simulink model "Production_ToBe_batched_upgrade1_run2026"  (R2025b)
settings: Solver=VariableStepAuto  StartTime=0.0  StopTime=105600  RelTol=1e-3
undefined symbols (not defined in the file or in its folder): m, n
(part 1 of 2)
settings Model: Creator=MSI  LastModifiedBy=MSI

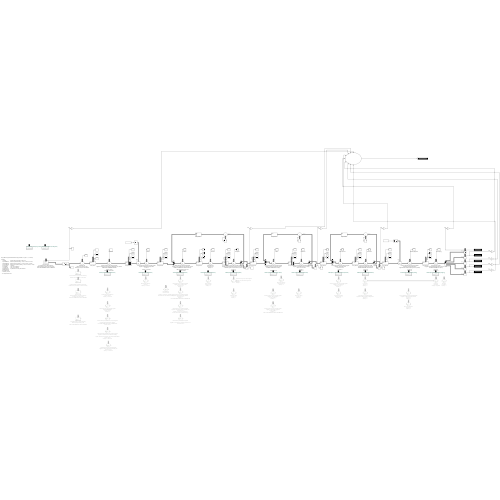
[thumbnail: Simulink's stored preview of the top-level diagram]
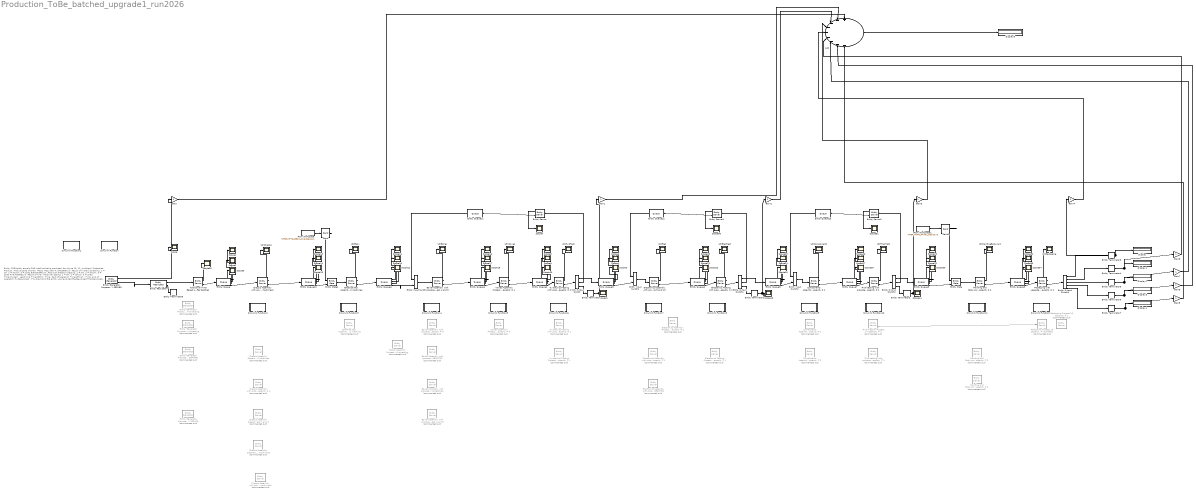
== system Production_ToBe_batched_upgrade1_run2026 ==
  note: Entity (ONE entity equals ONE machine being produced, be it type 10, 11, or others.)
      |
      | Properties:
      | Product : Product code of entity (PC10, PC11 etc)
      | HydTestResult : Result of hydraulics testing. 1 = OK, 2 = rework, 3 = scrap
      | ElecTestResult : Result of electronic testing. 1 = OK, 2 = rework, 3 = scrap
      | FinalTestResult : Result of final (machine) testing. 1 = OK, 2 = rework, 3 = scrap
      | TimeinSytem : Lead time
      | TimeAtStart : Time, start of operation
      | TimeAtFinish : Time, end of operation
      | HydReworked : If hydraulics of the entity was reworked
      | ElecReworked
      | FinalReworked
      | Endtime, process
      | TTP, process for each
  Add : Sum  Inputs=+--------
  Additional Time Based on the last entity type Models the setup time after batches : EntityServer  InputPortMessageModes=m  OutputPortMessageModes=n,m  Capacity=1  ServiceTimeSource=MATLAB action  ServiceTimeAction=|  Utilization=on
      | % Since this server is a proxy, dt = 0
      | dt = 0;
      | 
      | % Setup times
      | persistent last_product;
      | 
      | if isempty(last_product)
      |     last_product = 0;
      | end
      | 
      | setuptime = 0;
      | 
      | if last_product == 0
      |     % First entity - no setup time needed
      |     setuptime = 0;
      | elseif last_product ~= entity.Product
      |     % Product change detected - apply setup time based on previous product
      |     if last_product == 1
      |         setuptime = 0;
      |     elseif last_product == 2
      |         setuptime = 0;
      |     elseif last_product == 3
      |         setuptime = 15;
      |     elseif last_product == 4
      |         setuptime = 30;
      |     else
      |         setuptime = 35;
      |     end
      | end
      | 
      | dt = dt + setuptime;
      | last_product = entity.Product;
      settings: OutputPortMap=o5,o9
  "Boiler Assembly Process 4 and 5 Capacity = 3 machines, operated by 3 Rework decision after hydraulics testing" : EntityServer  Commented=on  InputPortMessageModes=m  OutputPortMessageModes=n,m  Capacity=3  ServiceTimeSource=MATLAB action  ServiceTimeAction=|  ServiceCompleteAction=|  Utilization=on
      ServiceTimeAction=|
      | % Main action of the server. Which means, this code explains what the entity department should be doing
      | % Assign entity processing times based on the time listed on the spreadsheet
      | % For process 4 and 5
      | 
      | generateTime = @(mu, cv) lognrnd(log(mu) - 0.5*log(1+cv^2), sqrt(log(1+cv^2)));
      | 
      | if entity.HydReworked == 1;
      |     dt = 1;
      | else
      |     if entity.Product == 1 | entity.Product == 3
      |     dt = generateTime(20.4, 1) + generateTime(19.9, 1);
      |     elseif entity.Product == 2 | entity.Product == 4 | entity.Product == 5
      |     dt = generateTime(28.2, 1) + generateTime (19.9, 1);
      |     else
      |     dt = 0; 
      |     end
      | end
      | 
      | % Setup times
      | persistent last_product;
      | 
      | if isempty(last_product)
      |     last_product = 0;
      | end
      | 
      | setuptime = 0;
      | 
      | if last_product == 0
      |     % First entity - no setup time needed
      |     setuptime = 0;
      | elseif last_product ~= entity.Product
      |     % Product change detected - apply setup time based on previous product
      |     if last_product == 1
      |         setuptime = 3;
      |     elseif last_product == 2
      |         setuptime = 4;
      |     elseif last_product == 3
      |         setuptime = 3;
      |     elseif last_product == 4
      |         setuptime = 4;
      |     else
      |         setuptime = 4;
      |     end
      | end
      | 
      | dt = dt + setuptime;
      | last_product = entity.Product;
      ServiceCompleteAction=|
      | % Define persistent variables to track the total throughput time and entity count
      | persistent TTPtotal entityCount;
      | % TTPtotal = tracks the total TTP of the system. In which, when every new station is visited, the time is added
      | % entityCount =
      | 
      | % Initialize the persistent variables if they are empty
      | if isempty(TTPtotal)
      |     TTPtotal = 0;
      | end
      | if isempty(entityCount)
      |     entityCount = 0;
      | end
      | 
      | % Read the current entity's final time
      | entity.EndTimeBoiler = ReadTime();
      | 
      | % Calculate the TTP for the chassis department for the specific entity
      | % INCLUDES wait time
      | entity.TTPboiler = abs(entity.EndTimeBoiler - entity.EndTimeEbox);
      | 
      | % Update the total throughput time and entity count
      | % This is done AFTER the process, 
      |     % to mark that the entity has gone through the chassis department 
      |         % (thus TTPchassis being added)
      |             % and add that the entity, for each entity after being processed
      |             
      | TTPtotal = TTPtotal + entity.TTPboiler;
      | entityCount = entityCount + 1;
      | 
      | % Calculate the average throughput time for the chassis department
      | avgTTPboiler = TTPtotal / entityCount;
      | 
      | % Send the average throughput time to the workspace
      | ToWorkspace_Boiler(avgTTPboiler);
      settings: OutputPortMap=o5,o9
  Boiler Assembly with proposed upgrade Upgrade = AR based assembly assistant Process 4 and 5 Capacity = 1 HAS TO BE PAIRED WITH ENTITY GENERATOR : EntityServer  Commented=on  InputPortMessageModes=m  OutputPortMessageModes=n,m  Capacity=3  ServiceTimeSource=MATLAB action  ServiceTimeAction=|  ServiceCompleteAction=|  Utilization=on
      ServiceTimeAction=|
      | % Main action of the server. Which means, this code explains what the entity department should be doing
      | % Assign entity processing times based on the time listed on the spreadsheet
      | % For process 4 and 5
      | 
      | generateTime = @(mu, cv) lognrnd(log(mu) - 0.5*log(1+cv^2), sqrt(log(1+cv^2)));
      | 
      | if entity.HydReworked == 1;
      |     dt = 1;
      | else
      |     if entity.Product == 10 | entity.Product == 11
      |     dt = generateTime(20.4, 1) + generateTime(19.9, 1);
      |     dt = dt * 0.9;
      |     elseif entity.Product == 20 | entity.Product == 21 | entity.Product == 35
      |     dt = generateTime(28.2, 1) + generateTime (19.9, 1);
      |     dt = dt * 0.9;
      |     else
      |     dt = 0; 
      |     end
      | end
      ServiceCompleteAction=|
      | % Define persistent variables to track the total throughput time and entity count
      | persistent TTPtotal entityCount;
      | % TTPtotal = tracks the total TTP of the system. In which, when every new station is visited, the time is added
      | % entityCount =
      | 
      | % Initialize the persistent variables if they are empty
      | if isempty(TTPtotal)
      |     TTPtotal = 0;
      | end
      | if isempty(entityCount)
      |     entityCount = 0;
      | end
      | 
      | % Read the current entity's final time
      | entity.EndTimeBoiler = ReadTime();
      | 
      | % Calculate the TTP for the chassis department for the specific entity
      | % INCLUDES wait time
      | entity.TTPboiler = abs(entity.EndTimeBoiler - entity.EndTimeEbox);
      | 
      | % Update the total throughput time and entity count
      | % This is done AFTER the process, 
      |     % to mark that the entity has gone through the chassis department 
      |         % (thus TTPchassis being added)
      |             % and add that the entity, for each entity after being processed
      |             
      | TTPtotal = TTPtotal + entity.TTPboiler;
      | entityCount = entityCount + 1;
      | 
      | % Calculate the average throughput time for the chassis department
      | avgTTPboiler = TTPtotal / entityCount;
      | 
      | % Send the average throughput time to the workspace
      | ToWorkspace_Boiler(avgTTPboiler);
      settings: OutputPortMap=o5,o9
  "Boiler Assembly with proposed upgrade Upgrade = Automated pressure regulation tool Process 4 and 5 Capacity = 3 machines, operated by 3 Rework decision after hydraulics testing1" : EntityServer  Commented=on  InputPortMessageModes=m  OutputPortMessageModes=n,m  Capacity=3  ServiceTimeSource=MATLAB action  ServiceTimeAction=|  ServiceCompleteAction=|  Utilization=on
      ServiceTimeAction=|
      | % Main action of the server. Which means, this code explains what the entity department should be doing
      | % Assign entity processing times based on the time listed on the spreadsheet
      | % For process 4 and 5
      | 
      | generateTime = @(mu, cv) lognrnd(log(mu) - 0.5*log(1+cv^2), sqrt(log(1+cv^2)));
      | 
      | if entity.HydReworked == 1;
      |     dt = 1;
      | else
      |     if entity.Product == 10 | entity.Product == 11
      |     dt = generateTime(20.4, 1) + generateTime(19.9, 1);
      |     dt = dt * 0.95;
      |     elseif entity.Product == 20 | entity.Product == 21 | entity.Product == 35
      |     dt = generateTime(28.2, 1) + generateTime (19.9, 1);
      |     dt = dt * 0.95;
      |     else
      |     dt = 0; 
      |     end
      | end
      ServiceCompleteAction=|
      | % Define persistent variables to track the total throughput time and entity count
      | persistent TTPtotal entityCount;
      | % TTPtotal = tracks the total TTP of the system. In which, when every new station is visited, the time is added
      | % entityCount =
      | 
      | % Initialize the persistent variables if they are empty
      | if isempty(TTPtotal)
      |     TTPtotal = 0;
      | end
      | if isempty(entityCount)
      |     entityCount = 0;
      | end
      | 
      | % Read the current entity's final time
      | entity.EndTimeBoiler = ReadTime();
      | 
      | % Calculate the TTP for the chassis department for the specific entity
      | % INCLUDES wait time
      | entity.TTPboiler = abs(entity.EndTimeBoiler - entity.EndTimeEbox);
      | 
      | % Update the total throughput time and entity count
      | % This is done AFTER the process, 
      |     % to mark that the entity has gone through the chassis department 
      |         % (thus TTPchassis being added)
      |             % and add that the entity, for each entity after being processed
      |             
      | TTPtotal = TTPtotal + entity.TTPboiler;
      | entityCount = entityCount + 1;
      | 
      | % Calculate the average throughput time for the chassis department
      | avgTTPboiler = TTPtotal / entityCount;
      | 
      | % Send the average throughput time to the workspace
      | ToWorkspace_Boiler(avgTTPboiler);
      settings: OutputPortMap=o5,o9
  Boiler Assembly with proposed upgrade Upgrade = Boiler insertion robot Process 4 and 5 Capacity = 3 : EntityServer  Commented=on  InputPortMessageModes=m  OutputPortMessageModes=n,m  Capacity=3  ServiceTimeSource=MATLAB action  ServiceTimeAction=|  ServiceCompleteAction=|  Utilization=on
      ServiceTimeAction=|
      | % Main action of the server. Which means, this code explains what the entity department should be doing
      | % Assign entity processing times based on the time listed on the spreadsheet
      | % For process 4 and 5
      | 
      | generateTime = @(mu, cv) lognrnd(log(mu) - 0.5*log(1+cv^2), sqrt(log(1+cv^2)));
      | 
      | if entity.HydReworked == 1;
      |     dt = 1;
      | else
      |     if entity.Product == 10 | entity.Product == 11
      |     dt = (generateTime(20.4, 1)) * 0.8 + generateTime(19.9, 1);
      |     elseif entity.Product == 20 | entity.Product == 21 | entity.Product == 35
      |     dt = (generateTime(28.2, 1)) * 0.85 + generateTime (19.9, 1);
      |     else
      |     dt = 0; 
      |     end
      | end
      ServiceCompleteAction=|
      | % Define persistent variables to track the total throughput time and entity count
      | persistent TTPtotal entityCount;
      | % TTPtotal = tracks the total TTP of the system. In which, when every new station is visited, the time is added
      | % entityCount =
      | 
      | % Initialize the persistent variables if they are empty
      | if isempty(TTPtotal)
      |     TTPtotal = 0;
      | end
      | if isempty(entityCount)
      |     entityCount = 0;
      | end
      | 
      | % Read the current entity's final time
      | entity.EndTimeBoiler = ReadTime();
      | 
      | % Calculate the TTP for the chassis department for the specific entity
      | % INCLUDES wait time
      | entity.TTPboiler = abs(entity.EndTimeBoiler - entity.EndTimeEbox);
      | 
      | % Update the total throughput time and entity count
      | % This is done AFTER the process, 
      |     % to mark that the entity has gone through the chassis department 
      |         % (thus TTPchassis being added)
      |             % and add that the entity, for each entity after being processed
      |             
      | TTPtotal = TTPtotal + entity.TTPboiler;
      | entityCount = entityCount + 1;
      | 
      | % Calculate the average throughput time for the chassis department
      | avgTTPboiler = TTPtotal / entityCount;
      | 
      | % Send the average throughput time to the workspace
      | ToWorkspace_Boiler(avgTTPboiler);
      settings: OutputPortMap=o5,o9
  Boiler Assembly with proposed upgrade Upgrade = Vision-guided robot for main boiler insertion DOUBLE UPGRADE with AR based assembly TRIPLE upgrade insertion robot Process 4 and 5 : EntityServer  InputPortMessageModes=m  OutputPortMessageModes=n,m  Capacity=3  ServiceTimeSource=MATLAB action  ServiceTimeAction=|  ServiceCompleteAction=|  Utilization=on
      ServiceTimeAction=|
      | % Main action of the server. Which means, this code explains what the entity department should be doing
      | % Assign entity processing times based on the time listed on the spreadsheet
      | % For process 4 and 5
      | 
      | generateTime = @(mu, cv) lognrnd(log(mu) - 0.5*log(1+cv^2), sqrt(log(1+cv^2)));
      | 
      | if entity.HydReworked == 1;
      |     dt = 1;
      | else
      |     if entity.Product == 1 | entity.Product == 2
      |     dt = generateTime(20.4, 1) + generateTime(19.9, 1); %triple upgrade
      |     dt = dt * 0.65;
      |     elseif entity.Product == 3 | entity.Product == 4 | entity.Product == 5
      |     dt = generateTime(28.2, 1) + generateTime (19.9, 1); %triple upgrade
      |     dt = dt * 0.65;
      |     else
      |     dt = 0; 
      |     end
      | end
      | 
      | % double upgrade
      | dt = dt * 0.9;
      | 
      | 
      | % Setup times
      | persistent last_product;
      | 
      | if isempty(last_product)
      |     last_product = 0;
      | end
      | 
      | setuptime = 0;
      | 
      | if last_product == 0
      |     % First entity - no setup time needed
      |     setuptime = 0;
      | elseif last_product ~= entity.Product
      |     % Product change detected - apply setup time based on previous product
      |     if last_product == 1
      |         setuptime = 3;
      |     elseif last_product == 2
      |         setuptime = 4;
      |     elseif last_product == 3
      |         setuptime = 3;
      |     elseif last_product == 4
      |         setuptime = 4;
      |     else
      |         setuptime = 4;
      |     end
      | end
      | 
      | dt = dt + setuptime;
      | last_product = entity.Product;
      ServiceCompleteAction=|
      | % Define persistent variables to track the total throughput time and entity count
      | persistent TTPtotal entityCount;
      | % TTPtotal = tracks the total TTP of the system. In which, when every new station is visited, the time is added
      | % entityCount =
      | 
      | % Initialize the persistent variables if they are empty
      | if isempty(TTPtotal)
      |     TTPtotal = 0;
      | end
      | if isempty(entityCount)
      |     entityCount = 0;
      | end
      | 
      | % Read the current entity's final time
      | entity.EndTimeBoiler = ReadTime();
      | 
      | % Calculate the TTP for the chassis department for the specific entity
      | % INCLUDES wait time
      | entity.TTPboiler = abs(entity.EndTimeBoiler - entity.EndTimeEbox);
      | 
      | % Update the total throughput time and entity count
      | % This is done AFTER the process, 
      |     % to mark that the entity has gone through the chassis department 
      |         % (thus TTPchassis being added)
      |             % and add that the entity, for each entity after being processed
      |             
      | TTPtotal = TTPtotal + entity.TTPboiler;
      | entityCount = entityCount + 1;
      | 
      | % Calculate the average throughput time for the chassis department
      | avgTTPboiler = TTPtotal / entityCount;
      | 
      | % Send the average throughput time to the workspace
      | ToWorkspace_Boiler(avgTTPboiler);
      settings: OutputPortMap=o5,o9
  "Boiler Assembly with proposed upgrade Upgrade = extra workbench, capacity grew from 3 to 4 Process 4 and 5" : EntityServer  Commented=on  InputPortMessageModes=m  OutputPortMessageModes=n,m  Capacity=4  ServiceTimeSource=MATLAB action  ServiceTimeAction=|  ServiceCompleteAction=|  Utilization=on
      ServiceTimeAction=|
      | % Main action of the server. Which means, this code explains what the entity department should be doing
      | % Assign entity processing times based on the time listed on the spreadsheet
      | % For process 4 and 5
      | 
      | generateTime = @(mu, cv) lognrnd(log(mu) - 0.5*log(1+cv^2), sqrt(log(1+cv^2)));
      | 
      | if entity.HydReworked == 1;
      |     dt = 1;
      | else
      |     if entity.Product == 10 | entity.Product == 11
      |     dt = generateTime(20.4, 1) + generateTime(19.9, 1);
      |     elseif entity.Product == 20 | entity.Product == 21 | entity.Product == 35
      |     dt = generateTime(28.2, 1) + generateTime (19.9, 1);
      |     else
      |     dt = 0; 
      |     end
      | end
      ServiceCompleteAction=|
      | % Define persistent variables to track the total throughput time and entity count
      | persistent TTPtotal entityCount;
      | % TTPtotal = tracks the total TTP of the system. In which, when every new station is visited, the time is added
      | % entityCount =
      | 
      | % Initialize the persistent variables if they are empty
      | if isempty(TTPtotal)
      |     TTPtotal = 0;
      | end
      | if isempty(entityCount)
      |     entityCount = 0;
      | end
      | 
      | % Read the current entity's final time
      | entity.EndTimeBoiler = ReadTime();
      | 
      | % Calculate the TTP for the chassis department for the specific entity
      | % INCLUDES wait time
      | entity.TTPboiler = abs(entity.EndTimeBoiler - entity.EndTimeEbox);
      | 
      | % Update the total throughput time and entity count
      | % This is done AFTER the process, 
      |     % to mark that the entity has gone through the chassis department 
      |         % (thus TTPchassis being added)
      |             % and add that the entity, for each entity after being processed
      |             
      | TTPtotal = TTPtotal + entity.TTPboiler;
      | entityCount = entityCount + 1;
      | 
      | % Calculate the average throughput time for the chassis department
      | avgTTPboiler = TTPtotal / entityCount;
      | 
      | % Send the average throughput time to the workspace
      | ToWorkspace_Boiler(avgTTPboiler);
      settings: OutputPortMap=o5,o9
  "Chassis Assembly Departmen with proposed upgrade Upgrade = Smart fixtures wth automatic clamping Impact = Assembly time variability -50%, ONLY GROUP HEAD Process 1 and 2 Capacity = 3 machines1" : EntityServer  Commented=on  InputPortMessageModes=m  OutputPortMessageModes=n,m  Capacity=3  ServiceTimeSource=MATLAB action  ServiceTimeAction=|  ServiceCompleteAction=|  Utilization=on
      ServiceTimeAction=|
      | % Main action of the server
      | 
      | % Function to generate processing time based on mean and CV using lognormal
      | generateTime = @(mu, cv) lognrnd(log(mu) - 0.5*log(1+cv^2), sqrt(log(1+cv^2)));
      | 
      | if entity.Product == 1
      |     dt = generateTime(29.7, 0.8) + generateTime(14.7, 0.4);
      | elseif entity.Product == 2
      |     dt = generateTime(31.2, 0.8) + generateTime(14.7, 0.4);
      | elseif entity.Product == 3
      |     dt = generateTime(29.7, 0.8) + generateTime(17.6, 0.4);
      | elseif entity.Product == 4
      |     dt = generateTime(31.2, 0.8) + generateTime(17.6, 0.4);
      | elseif entity.Product == 5
      |     dt = generateTime(34.4, 0.8) + generateTime(17.6, 0.4);
      | else
      |     dt = 0; 
      | end
      | 
      | % Setup times
      | persistent last_product;
      | last_product = 0;
      | setuptime = 0;
      | if last_product == 0
      |     last_product = entity.Product;   % first entity
      |     dt = dt + setuptime;
      | else
      |     if last_product == entity.Product;
      |         dt = dt + setuptime;
      |     else
      |         if last_product ~= entity.Product
      |             if last_product == 1
      |                 setuptime = 5;
      |                 dt = dt + setuptime;
      |             elseif last_product == 2
      |                 setuptime = 6;
      |                 dt = dt + setuptime;
      |             elseif last_product == 3
      |                 setuptime = 5;
      |                 dt = dt + setuptime;
      |             elseif last_product == 4
      |                 setuptime = 6;
      |                 dt = dt + setuptime;
      |             else
      |                 setuptime = 6;
      |                 dt = dt + setuptime;
      |             end
      |         end
      |     end
      |     last_product = entity.Product;
      | end
      ServiceCompleteAction=|
      | % Define persistent variables to track the total throughput time and entity count
      | persistent TTPtotal entityCount;
      | % TTPtotal = tracks the total TTP of the system. In which, when every new station is visited, the time is added
      | % entityCount =
      | 
      | % Initialize the persistent variables if they are empty
      | if isempty(TTPtotal)
      |     TTPtotal = 0;
      | end
      | if isempty(entityCount)
      |     entityCount = 0;
      | end
      | 
      | % Read the current entity's final time
      | entity.EndTimeChassis = ReadTime();
      | 
      | % Calculate the TTP for the chassis department for the specific entity
      | % INCLUDES wait time
      | entity.TTPchassis = abs(entity.EndTimeChassis - entity.StartTime);
      | 
      | % Update the total throughput time and entity count
      | % This is done AFTER the process, 
      |     % to mark that the entity has gone through the chassis department 
      |         % (thus TTPchassis being added)
      |             % and add that the entity, for each entity after being processed
      |             
      | TTPtotal = TTPtotal + entity.TTPchassis;
      | entityCount = entityCount + 1;
      | 
      | % Calculate the average throughput time for the chassis department
      | avgTTPchassis = TTPtotal / entityCount;
      | 
      | % Send the average throughput time to the workspace
      | ToWorkspace_Chassis(avgTTPchassis);
      settings: OutputPortMap=o5,o9
  Chassis Assembly Department Process 1 and 2 Capacity = 3 machines : EntityServer  Commented=on  InputPortMessageModes=m  OutputPortMessageModes=n,m  Capacity=3  ServiceTimeSource=MATLAB action  ServiceTimeAction=|  ServiceCompleteAction=|  Utilization=on
      ServiceTimeAction=|
      | % Main action of the server
      | 
      | % Function to generate processing time based on mean and CV using lognormal
      | generateTime = @(mu, cv) lognrnd(log(mu) - 0.5*log(1+cv^2), sqrt(log(1+cv^2)));
      | 
      | if entity.Product == 1
      |     dt = generateTime(29.7, 0.8) + generateTime(14.7, 0.8);
      | elseif entity.Product == 2
      |     dt = generateTime(31.2, 0.8) + generateTime(14.7, 0.8);
      | elseif entity.Product == 3
      |     dt = generateTime(29.7, 0.8) + generateTime(17.6, 0.8);
      | elseif entity.Product == 4
      |     dt = generateTime(31.2, 0.8) + generateTime(17.6, 0.8);
      | elseif entity.Product == 5
      |     dt = generateTime(34.4, 0.8) + generateTime(17.6, 0.8);
      | else
      |     dt = 0; 
      | end
      | 
      | % Setup times
      | persistent last_product;
      | 
      | if isempty(last_product)
      |     last_product = 0;
      | end
      | 
      | setuptime = 0;
      | 
      | if last_product == 0
      |     % First entity - no setup time needed
      |     setuptime = 0;
      | elseif last_product ~= entity.Product
      |     % Product change detected - apply setup time based on previous product
      |     if last_product == 1
      |         setuptime = 5;
      |     elseif last_product == 2
      |         setuptime = 6;
      |     elseif last_product == 3
      |         setuptime = 5;
      |     elseif last_product == 4
      |         setuptime = 6;
      |     else
      |         setuptime = 6;
      |     end
      | end
      | 
      | dt = dt + setuptime;
      | last_product = entity.Product;
      ServiceCompleteAction=|
      | % Define persistent variables to track the total throughput time and entity count
      | persistent TTPtotal entityCount;
      | % TTPtotal = tracks the total TTP of the system. In which, when every new station is visited, the time is added
      | % entityCount =
      | 
      | % Initialize the persistent variables if they are empty
      | if isempty(TTPtotal)
      |     TTPtotal = 0;
      | end
      | if isempty(entityCount)
      |     entityCount = 0;
      | end
      | 
      | % Read the current entity's final time
      | entity.EndTimeChassis = ReadTime();
      | 
      | % Calculate the TTP for the chassis department for the specific entity
      | % INCLUDES wait time
      | entity.TTPchassis = abs(entity.EndTimeChassis - entity.StartTime);
      | 
      | % Update the total throughput time and entity count
      | % This is done AFTER the process, 
      |     % to mark that the entity has gone through the chassis department 
      |         % (thus TTPchassis being added)
      |             % and add that the entity, for each entity after being processed
      |             
      | TTPtotal = TTPtotal + entity.TTPchassis;
      | entityCount = entityCount + 1;
      | 
      | % Calculate the average throughput time for the chassis department
      | avgTTPchassis = TTPtotal / entityCount;
      | 
      | % Send the average throughput time to the workspace
      | ToWorkspace_Chassis(avgTTPchassis);
      settings: OutputPortMap=o5,o9
  Chassis Assembly Department with proposed upgrade Upgrade= AR based assembly assistant HAS TO BE PAIRED WITH ENTITY GENERATOR Process 1 and 2 : EntityServer  Commented=on  InputPortMessageModes=m  OutputPortMessageModes=n,m  Capacity=3  ServiceTimeSource=MATLAB action  ServiceTimeAction=|  ServiceCompleteAction=|  Utilization=on
      ServiceTimeAction=|
      | % Main action of the server
      | 
      | % Function to generate processing time based on mean and CV using lognormal
      | generateTime = @(mu, cv) lognrnd(log(mu) - 0.5*log(1+cv^2), sqrt(log(1+cv^2)));
      | 
      | if entity.Product == 10
      |     dt = generateTime(29.7, 0.8) + generateTime(14.7, 0.8);
      |     dt = dt * 0.9;
      | elseif entity.Product == 20
      |     dt = generateTime(31.2, 0.8) + generateTime(14.7, 0.8);
      |     dt = dt * 0.9;
      | elseif entity.Product == 11
      |     dt = generateTime(29.7, 0.8) + generateTime(17.6, 0.8);
      |     dt = dt * 0.9;
      | elseif entity.Product == 21
      |     dt = generateTime(31.2, 0.8) + generateTime(17.6, 0.8);
      |     dt = dt * 0.9;
      | elseif entity.Product == 35
      |     dt = generateTime(34.4, 0.8) + generateTime(17.6, 0.8);
      |     dt = dt * 0.9;
      | else
      |     dt = 0; 
      | end
      ServiceCompleteAction=|
      | % Define persistent variables to track the total throughput time and entity count
      | persistent TTPtotal entityCount;
      | % TTPtotal = tracks the total TTP of the system. In which, when every new station is visited, the time is added
      | % entityCount =
      | 
      | % Initialize the persistent variables if they are empty
      | if isempty(TTPtotal)
      |     TTPtotal = 0;
      | end
      | if isempty(entityCount)
      |     entityCount = 0;
      | end
      | 
      | % Read the current entity's final time
      | entity.EndTimeChassis = ReadTime();
      | 
      | % Calculate the TTP for the chassis department for the specific entity
      | % INCLUDES wait time
      | entity.TTPchassis = abs(entity.EndTimeChassis - entity.StartTime);
      | 
      | % Update the total throughput time and entity count
      | % This is done AFTER the process, 
      |     % to mark that the entity has gone through the chassis department 
      |         % (thus TTPchassis being added)
      |             % and add that the entity, for each entity after being processed
      |             
      | TTPtotal = TTPtotal + entity.TTPchassis;
      | entityCount = entityCount + 1;
      | 
      | % Calculate the average throughput time for the chassis department
      | avgTTPchassis = TTPtotal / entityCount;
      | 
      | % Send the average throughput time to the workspace
      | ToWorkspace_Chassis(avgTTPchassis);
      settings: OutputPortMap=o5,o9
  Chassis Assembly with proposed upgrade EXTRA WORKBENCH Process 1 and 2 Capacity = 4 : EntityServer  Commented=on  InputPortMessageModes=m  OutputPortMessageModes=n,m  Capacity=4  ServiceTimeSource=MATLAB action  ServiceTimeAction=|  ServiceCompleteAction=|  Utilization=on
      ServiceTimeAction=|
      | % Main action of the server
      | 
      | % Function to generate processing time based on mean and CV using lognormal
      | generateTime = @(mu, cv) lognrnd(log(mu) - 0.5*log(1+cv^2), sqrt(log(1+cv^2)));
      | 
      | if entity.Product == 10
      |     dt = generateTime(29.7, 0.8) + generateTime(14.7, 0.8);
      | elseif entity.Product == 20
      |     dt = generateTime(31.2, 0.8) + generateTime(14.7, 0.8);
      | elseif entity.Product == 11
      |     dt = generateTime(29.7, 0.8) + generateTime(17.6, 0.8);
      | elseif entity.Product == 21
      |     dt = generateTime(31.2, 0.8) + generateTime(17.6, 0.8);
      | elseif entity.Product == 35
      |     dt = generateTime(34.4, 0.8) + generateTime(17.6, 0.8);
      | else
      |     dt = 0; 
      | end
      ServiceCompleteAction=|
      | % Define persistent variables to track the total throughput time and entity count
      | persistent TTPtotal entityCount;
      | % TTPtotal = tracks the total TTP of the system. In which, when every new station is visited, the time is added
      | % entityCount =
      | 
      | % Initialize the persistent variables if they are empty
      | if isempty(TTPtotal)
      |     TTPtotal = 0;
      | end
      | if isempty(entityCount)
      |     entityCount = 0;
      | end
      | 
      | % Read the current entity's final time
      | entity.EndTimeChassis = ReadTime();
      | 
      | % Calculate the TTP for the chassis department for the specific entity
      | % INCLUDES wait time
      | entity.TTPchassis = abs(entity.EndTimeChassis - entity.StartTime);
      | 
      | % Update the total throughput time and entity count
      | % This is done AFTER the process, 
      |     % to mark that the entity has gone through the chassis department 
      |         % (thus TTPchassis being added)
      |             % and add that the entity, for each entity after being processed
      |             
      | TTPtotal = TTPtotal + entity.TTPchassis;
      | entityCount = entityCount + 1;
      | 
      | % Calculate the average throughput time for the chassis department
      | avgTTPchassis = TTPtotal / entityCount;
      | 
      | % Send the average throughput time to the workspace
      | ToWorkspace_Chassis(avgTTPchassis);
      settings: OutputPortMap=o5,o9
  Chassis Assembly with proposed upgrade Upgrade = Group head precision assembly cell Process 1 and 2 Capacity = 3 machines1 : EntityServer  Commented=on  InputPortMessageModes=m  OutputPortMessageModes=n,m  Capacity=3  ServiceTimeSource=MATLAB action  ServiceTimeAction=|  ServiceCompleteAction=|  Utilization=on
      ServiceTimeAction=|
      | % Main action of the server
      | 
      | % Function to generate processing time based on mean and CV using lognormal
      | generateTime = @(mu, cv) lognrnd(log(mu) - 0.5*log(1+cv^2), sqrt(log(1+cv^2)));
      | 
      | if entity.Product == 10
      |     dt = generateTime(29.7, 0.8) + generateTime(14.7, 0.8) * 0.7;
      | elseif entity.Product == 20
      |     dt = generateTime(31.2, 0.8) + generateTime(14.7, 0.8) * 0.7;
      | elseif entity.Product == 11
      |     dt = generateTime(29.7, 0.8) + generateTime(17.6, 0.8) * 0.7;
      | elseif entity.Product == 21
      |     dt = generateTime(31.2, 0.8) + generateTime(17.6, 0.8) * 0.7;
      | elseif entity.Product == 35
      |     dt = generateTime(34.4, 0.8) + generateTime(17.6, 0.8) * 0.7;
      | else
      |     dt = 0; 
      | end
      | 
      | % Setup times
      | persistent last_product;
      | 
      | if isempty(last_product)
      |     last_product = 0;
      | end
      | 
      | setuptime = 0;
      | 
      | if last_product == 0
      |     % First entity - no setup time needed
      |     setuptime = 0;
      | elseif last_product ~= entity.Product
      |     % Product change detected - apply setup time based on previous product
      |     if last_product == 1
      |         setuptime = 5;
      |     elseif last_product == 2
      |         setuptime = 6;
      |     elseif last_product == 3
      |         setuptime = 5;
      |     elseif last_product == 4
      |         setuptime = 6;
      |     else
      |         setuptime = 6;
      |     end
      | end
      | 
      | dt = dt + setuptime;
      | last_product = entity.Product;
      ServiceCompleteAction=|
      | % Define persistent variables to track the total throughput time and entity count
      | persistent TTPtotal entityCount;
      | % TTPtotal = tracks the total TTP of the system. In which, when every new station is visited, the time is added
      | % entityCount =
      | 
      | % Initialize the persistent variables if they are empty
      | if isempty(TTPtotal)
      |     TTPtotal = 0;
      | end
      | if isempty(entityCount)
      |     entityCount = 0;
      | end
      | 
      | % Read the current entity's final time
      | entity.EndTimeChassis = ReadTime();
      | 
      | % Calculate the TTP for the chassis department for the specific entity
      | % INCLUDES wait time
      | entity.TTPchassis = abs(entity.EndTimeChassis - entity.StartTime);
      | 
      | % Update the total throughput time and entity count
      | % This is done AFTER the process, 
      |     % to mark that the entity has gone through the chassis department 
      |         % (thus TTPchassis being added)
      |             % and add that the entity, for each entity after being processed
      |             
      | TTPtotal = TTPtotal + entity.TTPchassis;
      | entityCount = entityCount + 1;
      | 
      | % Calculate the average throughput time for the chassis department
      | avgTTPchassis = TTPtotal / entityCount;
      | 
      | % Send the average throughput time to the workspace
      | ToWorkspace_Chassis(avgTTPchassis);
      settings: OutputPortMap=o5,o9
  Chassis Assembly with proposed upgrade Upgrade = collaborative robot with force feedback for main chassis ADDITIONAL WORKBENCH ADDED Process 1 and 2 Capacity = 3 machines1 : EntityServer  InputPortMessageModes=m  OutputPortMessageModes=n,m  Capacity=3  ServiceTimeSource=MATLAB action  ServiceTimeAction=|  ServiceCompleteAction=|  Utilization=on
      ServiceTimeAction=|
      | % Main action of the server
      | 
      | % Function to generate processing time based on mean and CV using lognormal
      | generateTime = @(mu, cv) lognrnd(log(mu) - 0.5*log(1+cv^2), sqrt(log(1+cv^2)));
      | 
      | if entity.Product == 1
      |     dt = generateTime(29.7, 0.8) * 0.8 + generateTime(14.7, 0.8);
      | elseif entity.Product == 3
      |     dt = generateTime(31.2, 0.8) * 0.8 + generateTime(14.7, 0.8);
      | elseif entity.Product == 2
      |     dt = generateTime(29.7, 0.8) * 0.8 + generateTime(17.6, 0.8);
      | elseif entity.Product == 4
      |     dt = generateTime(31.2, 0.8) * 0.8 + generateTime(17.6, 0.8);
      | elseif entity.Product == 5
      |     dt = generateTime(34.4, 0.8) * 0.8 + generateTime(17.6, 0.8);
      | else
      |     dt = 0; 
      | end
      ServiceCompleteAction=|
      | % Define persistent variables to track the total throughput time and entity count
      | persistent TTPtotal entityCount;
      | % TTPtotal = tracks the total TTP of the system. In which, when every new station is visited, the time is added
      | % entityCount =
      | 
      | % Initialize the persistent variables if they are empty
      | if isempty(TTPtotal)
      |     TTPtotal = 0;
      | end
      | if isempty(entityCount)
      |     entityCount = 0;
      | end
      | 
      | % Read the current entity's final time
      | entity.EndTimeChassis = ReadTime();
      | 
      | % Calculate the TTP for the chassis department for the specific entity
      | % INCLUDES wait time
      | entity.TTPchassis = abs(entity.EndTimeChassis - entity.StartTime);
      | 
      | % Update the total throughput time and entity count
      | % This is done AFTER the process, 
      |     % to mark that the entity has gone through the chassis department 
      |         % (thus TTPchassis being added)
      |             % and add that the entity, for each entity after being processed
      |             
      | TTPtotal = TTPtotal + entity.TTPchassis;
      | entityCount = entityCount + 1;
      | 
      | % Calculate the average throughput time for the chassis department
      | avgTTPchassis = TTPtotal / entityCount;
      | 
      | % Send the average throughput time to the workspace
      | ToWorkspace_Chassis(avgTTPchassis);
      settings: OutputPortMap=o5,o9
  Components Assembly Process 12 and 13 Capacity = 2 : EntityServer  Commented=on  InputPortMessageModes=m  OutputPortMessageModes=n,m  Capacity=2  ServiceTimeSource=MATLAB action  ServiceTimeValue=32  ServiceTimeAction=|  ServiceCompleteAction=|  Utilization=on
      | generateTime = @(mu, cv) lognrnd(log(mu) - 0.5*log(1+cv^2), sqrt(log(1+cv^2)));
      | 
      | if entity.FinalReworked == 1;
      |     dt = 1;
      | else
      |     if entity.Product == 1
      |     dt = generateTime (11.7, 0.3) + generateTime (14.3, 0.3);
      |     elseif entity.Product == 2
      |     dt = generateTime (14.3, 0.3) + generateTime (13, 0.3) + generateTime(13, 0.3);
      |     elseif entity.Product == 3
      |     dt = generateTime (7.8, 0.3) + generateTime (13, 0.3) + generateTime(19.5, 0.3);
      |     elseif entity.Product == 4
      |     dt = generateTime (9.1, 0.3) + generateTime (13, 0.3) + generateTime(22.1, 0.3);
      |     elseif entity.Product == 5
      |     dt = generateTime (18.2, 0.3) + generateTime (11.7, 0.3) + generateTime(22.1, 0.3);
      |     else
      |     dt = 0;
      |     end
      | end
      | 
      | % Setup times
      | persistent last_product;
      | 
      | if isempty(last_product)
      |     last_product = 0;
      | end
      | 
      | setuptime = 0;
      | 
      | if last_product == 0
      |     % First entity - no setup time needed
      |     setuptime = 0;
      | elseif last_product ~= entity.Product
      |     % Product change detected - apply setup time based on previous product
      |     if last_product == 1
      |         setuptime = 1.5;
      |     else
      |         setuptime = 2;
      |     end
      | end
      | 
      | dt = dt + setuptime;
      | last_product = entity.Product;
      | % Define persistent variables to track the total throughput time and entity count
      | persistent TTPtotal entityCount;
      | % TTPtotal = tracks the total TTP of the system. In which, when every new station is visited, the time is added
      | % entityCount =
      | 
      | % Initialize the persistent variables if they are empty
      | if isempty(TTPtotal)
      |     TTPtotal = 0;
      | end
      | if isempty(entityCount)
      |     entityCount = 0;
      | end
      | 
      | % Read the current entity's final time
      | entity.EndTimeComponents = ReadTime();
      | 
      | % Calculate the TTP for the chassis department for the specific entity
      | % INCLUDES wait time
      | entity.TTPcomponents = abs(entity.EndTimeComponents - entity.EndTimeElecTest);
      | 
      | % Update the total throughput time and entity count
      | % This is done AFTER the process, 
      |     % to mark that the entity has gone through the chassis department 
      |         % (thus TTPchassis being added)
      |             % and add that the entity, for each entity after being processed
      |             
      | TTPtotal = TTPtotal + entity.TTPcomponents;
      | entityCount = entityCount + 1;
      | 
      | % Calculate the average throughput time for the chassis department
      | avgTTPcomponents = TTPtotal / entityCount;
      | 
      | % Send the average throughput time to the workspace
      | ToWorkspace_Components(avgTTPcomponents);
      settings: OutputPortMap=o5,o9
  Components Assembly with proposed upgrade Upgrade = collaborative robot Process 12 and 13 Capacity = 1 : EntityServer  InputPortMessageModes=m  OutputPortMessageModes=n,m  Capacity=2  ServiceTimeSource=MATLAB action  ServiceTimeValue=32  ServiceTimeAction=|  ServiceCompleteAction=|  Utilization=on
      | generateTime = @(mu, cv) lognrnd(log(mu) - 0.5*log(1+cv^2), sqrt(log(1+cv^2)));
      | 
      | if entity.FinalReworked == 1;
      |     dt = 1;
      | else
      |     if entity.Product == 1
      |     dt = generateTime (11.7, 0.3) + generateTime (14.3, 0.3);
      |     dt = dt * 0.7;
      |     elseif entity.Product == 3
      |     dt = generateTime (14.3, 0.3) + generateTime (13, 0.3) + generateTime(13, 0.3);
      |     dt = dt * 0.7;
      |     elseif entity.Product == 2
      |     dt = generateTime (7.8, 0.3) + generateTime (13, 0.3) + generateTime(19.5, 0.3);
      |     dt = dt * 0.7;
      |     elseif entity.Product == 4
      |     dt = generateTime (9.1, 0.3) + generateTime (13, 0.3) + generateTime(22.1, 0.3);
      |     dt = dt * 0.7;
      |     elseif entity.Product == 5
      |     dt = generateTime (18.2, 0.3) + generateTime (11.7, 0.3) + generateTime(22.1, 0.3);
      |     dt = dt * 0.7;
      |     else
      |     dt = 0;
      |     end
      | end
      | 
      | % Setup times
      | persistent last_product;
      | 
      | if isempty(last_product)
      |     last_product = 0;
      | end
      | 
      | setuptime = 0;
      | 
      | if last_product == 0
      |     % First entity - no setup time needed
      |     setuptime = 0;
      | elseif last_product ~= entity.Product
      |     % Product change detected - apply setup time based on previous product
      |     if last_product == 1
      |         setuptime = 1.5;
      |     else
      |         setuptime = 2;
      |     end
      | end
      | 
      | dt = dt + setuptime;
      | last_product = entity.Product;
      | % Define persistent variables to track the total throughput time and entity count
      | persistent TTPtotal entityCount;
      | % TTPtotal = tracks the total TTP of the system. In which, when every new station is visited, the time is added
      | % entityCount =
      | 
      | % Initialize the persistent variables if they are empty
      | if isempty(TTPtotal)
      |     TTPtotal = 0;
      | end
      | if isempty(entityCount)
      |     entityCount = 0;
      | end
      | 
      | % Read the current entity's final time
      | entity.EndTimeComponents = ReadTime();
      | 
      | % Calculate the TTP for the chassis department for the specific entity
      | % INCLUDES wait time
      | entity.TTPcomponents = abs(entity.EndTimeComponents - entity.EndTimeElecTest);
      | 
      | % Update the total throughput time and entity count
      | % This is done AFTER the process, 
      |     % to mark that the entity has gone through the chassis department 
      |         % (thus TTPchassis being added)
      |             % and add that the entity, for each entity after being processed
      |             
      | TTPtotal = TTPtotal + entity.TTPcomponents;
      | entityCount = entityCount + 1;
      | 
      | % Calculate the average throughput time for the chassis department
      | avgTTPcomponents = TTPtotal / entityCount;
      | 
      | % Send the average throughput time to the workspace
      | ToWorkspace_Components(avgTTPcomponents);
      settings: OutputPortMap=o5,o9
  Components Assembly with proposed upgrade Upgrade = extra workbench Process 12 and 13 Capacity = 1 : EntityServer  Commented=on  InputPortMessageModes=m  OutputPortMessageModes=n,m  Capacity=3  ServiceTimeSource=MATLAB action  ServiceTimeValue=32  ServiceTimeAction=|  ServiceCompleteAction=|  Utilization=on
      | generateTime = @(mu, cv) lognrnd(log(mu) - 0.5*log(1+cv^2), sqrt(log(1+cv^2)));
      | 
      | if entity.FinalReworked == 1;
      |     dt = 1;
      | else
      |     if entity.Product == 10
      |     dt = generateTime (11.7, 0.3) + generateTime (14.3, 0.3);
      |     elseif entity.Product == 20
      |     dt = generateTime (14.3, 0.3) + generateTime (13, 0.3) + generateTime(13, 0.3);
      |     elseif entity.Product == 11
      |     dt = generateTime (7.8, 0.3) + generateTime (13, 0.3) + generateTime(19.5, 0.3);
      |     elseif entity.Product == 21
      |     dt = generateTime (9.1, 0.3) + generateTime (13, 0.3) + generateTime(22.1, 0.3);
      |     elseif entity.Product == 35
      |     dt = generateTime (18.2, 0.3) + generateTime (11.7, 0.3) + generateTime(22.1, 0.3);
      |     else
      |     dt = 0;
      |     end
      | end
      | % Define persistent variables to track the total throughput time and entity count
      | persistent TTPtotal entityCount;
      | % TTPtotal = tracks the total TTP of the system. In which, when every new station is visited, the time is added
      | % entityCount =
      | 
      | % Initialize the persistent variables if they are empty
      | if isempty(TTPtotal)
      |     TTPtotal = 0;
      | end
      | if isempty(entityCount)
      |     entityCount = 0;
      | end
      | 
      | % Read the current entity's final time
      | entity.EndTimeComponents = ReadTime();
      | 
      | % Calculate the TTP for the chassis department for the specific entity
      | % INCLUDES wait time
      | entity.TTPcomponents = abs(entity.EndTimeComponents - entity.EndTimeElecTest);
      | 
      | % Update the total throughput time and entity count
      | % This is done AFTER the process, 
      |     % to mark that the entity has gone through the chassis department 
      |         % (thus TTPchassis being added)
      |             % and add that the entity, for each entity after being processed
      |             
      | TTPtotal = TTPtotal + entity.TTPcomponents;
      | entityCount = entityCount + 1;
      | 
      | % Calculate the average throughput time for the chassis department
      | avgTTPcomponents = TTPtotal / entityCount;
      | 
      | % Send the average throughput time to the workspace
      | ToWorkspace_Components(avgTTPcomponents);
      settings: OutputPortMap=o5,o9
  Display{,1..5} (6 alike) : Display
  Electrical Box Assembly Process 3 Capacity = 2 machine : EntityServer  Commented=on  InputPortMessageModes=m  OutputPortMessageModes=n,m  Capacity=2  ServiceTimeSource=MATLAB action  ServiceTimeValue=32  ServiceTimeAction=|  ServiceCompleteAction=|  Utilization=on
      ServiceTimeAction=|
      | % Process times
      | dt = 32;
      | 
      | % Setup times
      | persistent last_product;
      | 
      | if isempty(last_product)
      |     last_product = 0;
      | end
      | 
      | setuptime = 0;
      | 
      | if last_product == 0
      |     % First entity - no setup time needed
      |     setuptime = 0;
      | elseif last_product ~= entity.Product
      |     % Product change detected - apply setup time based on previous product
      |     setuptime = 4;
      | end
      | 
      | dt = dt + setuptime;
      | last_product = entity.Product;
      ServiceCompleteAction=|
      | % Define persistent variables to track the total throughput time and entity count
      | persistent TTPtotal entityCount;
      | % TTPtotal = tracks the total TTP of the system. In which, when every new station is visited, the time is added
      | % entityCount =
      | 
      | % Initialize the persistent variables if they are empty
      | if isempty(TTPtotal)
      |     TTPtotal = 0;
      | end
      | if isempty(entityCount)
      |     entityCount = 0;
      | end
      | 
      | % Read the current entity's final time
      | entity.EndTimeEbox = ReadTime();
      | 
      | % Calculate the TTP for the chassis department for the specific entity
      | % INCLUDES wait time
      | entity.TTPebox = abs(entity.EndTimeEbox - entity.EndTimeChassis);
      | 
      | % Update the total throughput time and entity count
      | % This is done AFTER the process, 
      |     % to mark that the entity has gone through the chassis department 
      |         % (thus TTPchassis being added)
      |             % and add that the entity, for each entity after being processed
      |             
      | TTPtotal = TTPtotal + entity.TTPebox;
      | entityCount = entityCount + 1;
      | 
      | % Calculate the average throughput time for the electrical box department
      | avgTTPebox = TTPtotal / entityCount;
      | 
      | % Send the average throughput time to the workspace
      | ToWorkspace_EBox(avgTTPebox);
      settings: OutputPortMap=o5,o9
  Electrical Box Assembly with proposed upgrade Upgrade = Additional assembly station Process 3 Capacity = 2 machine1 : EntityServer  InputPortMessageModes=m  OutputPortMessageModes=n,m  Capacity=3  ServiceTimeSource=MATLAB action  ServiceTimeValue=32  ServiceTimeAction=|  ServiceCompleteAction=|  Utilization=on
      ServiceTimeAction=|
      | dt = 32;
      | 
      | % Setup times
      | persistent last_product;
      | 
      | if isempty(last_product)
      |     last_product = 0;
      | end
      | 
      | setuptime = 0;
      | 
      | if last_product == 0
      |     % First entity - no setup time needed
      |     setuptime = 0;
      | elseif last_product ~= entity.Product
      |     % Product change detected - apply setup time based on previous product
      |     setuptime = 4;
      | end
      | 
      | dt = dt + setuptime;
      | last_product = entity.Product;
      ServiceCompleteAction=|
      | % Define persistent variables to track the total throughput time and entity count
      | persistent TTPtotal entityCount;
      | % TTPtotal = tracks the total TTP of the system. In which, when every new station is visited, the time is added
      | % entityCount =
      | 
      | % Initialize the persistent variables if they are empty
      | if isempty(TTPtotal)
      |     TTPtotal = 0;
      | end
      | if isempty(entityCount)
      |     entityCount = 0;
      | end
      | 
      | % Read the current entity's final time
      | entity.EndTimeEbox = ReadTime();
      | 
      | % Calculate the TTP for the chassis department for the specific entity
      | % INCLUDES wait time
      | entity.TTPebox = abs(entity.EndTimeEbox - entity.EndTimeChassis);
      | 
      | % Update the total throughput time and entity count
      | % This is done AFTER the process, 
      |     % to mark that the entity has gone through the chassis department 
      |         % (thus TTPchassis being added)
      |             % and add that the entity, for each entity after being processed
      |             
      | TTPtotal = TTPtotal + entity.TTPebox;
      | entityCount = entityCount + 1;
      | 
      | % Calculate the average throughput time for the electrical box department
      | avgTTPebox = TTPtotal / entityCount;
      | 
      | % Send the average throughput time to the workspace
      | ToWorkspace_EBox(avgTTPebox);
      settings: OutputPortMap=o5,o9
  Electronics Assembly Process 9 and 10 Capacity = 2 : EntityServer  Commented=on  InputPortMessageModes=m  OutputPortMessageModes=n,m  Capacity=2  ServiceTimeSource=MATLAB action  ServiceTimeValue=32  ServiceTimeAction=|  ServiceCompleteAction=|  Utilization=on
      | generateTime = @(mu, cv) lognrnd(log(mu) - 0.5*log(1+cv^2), sqrt(log(1+cv^2)));
      | 
      | if entity.ElecReworked == 1
      |     dt = 1;
      | else
      |     if entity.Product == 1
      |     dt = generateTime(10.4, 0.55) + generateTime(20.8, 0.55);
      |     elseif entity.Product == 2
      |     dt = generateTime (10.4, 0.55) + generateTime(25.1, 0.55);
      |     elseif entity.Product == 3 | entity.Product == 5
      |     dt = generateTime (12.1, 0.55) + generateTime (20.8, 0.55);
      |     elseif entity.Product == 4
      |     dt = generateTime (12.1, 0.55) + generateTime (25.1, 0.55);
      |     else
      |     dt = 0;
      |     end
      | end
      | 
      | % Setup times
      | persistent last_product;
      | 
      | if isempty(last_product)
      |     last_product = 0;
      | end
      | 
      | setuptime = 0;
      | 
      | if last_product == 0
      |     % First entity - no setup time needed
      |     setuptime = 0;
      | elseif last_product ~= entity.Product
      |     % Product change detected - apply setup time based on previous product
      |     setuptime = 2.5;
      | end
      | 
      | dt = dt + setuptime;
      | last_product = entity.Product;
      | % Define persistent variables to track the total throughput time and entity count
      | persistent TTPtotal entityCount;
      | 
      | % Initialize the persistent variables if they are empty
      | if isempty(TTPtotal)
      |     TTPtotal = 0;
      | end
      | if isempty(entityCount)
      |     entityCount = 0;
      | end
      | 
      | % Read the current entity's final time and calculate throughput time
      | entity.EndTimeElec = ReadTime();
      | entity.TTPelec = abs(entity.EndTimeElec - entity.EndTimeHydTest);
      | 
      | % Update the total throughput time and entity count
      | TTPtotal = TTPtotal + entity.TTPelec;
      | entityCount = entityCount + 1;
      | 
      | % Calculate the average throughput time
      | avgTTPelec = TTPtotal / entityCount;
      | 
      | % Send the average throughput time to the workspace
      | ToWorkspace_ElecAssembly(avgTTPelec);
      settings: OutputPortMap=o5,o9
  Electronics Assembly with proposed upgrade Upgrade = CPU testing intelligence Process 9 and 10 Capacity = 1 HAS TO BE PAIRED WITH ENTITY GENERATOR : EntityServer  Commented=on  InputPortMessageModes=m  OutputPortMessageModes=n,m  Capacity=2  ServiceTimeSource=MATLAB action  ServiceTimeValue=32  ServiceTimeAction=|  ServiceCompleteAction=|  Utilization=on
      | generateTime = @(mu, cv) lognrnd(log(mu) - 0.5*log(1+cv^2), sqrt(log(1+cv^2)));
      | 
      | if entity.ElecReworked == 1
      |     dt = 1;
      | else
      |     if entity.Product == 10
      |     dt = generateTime(10.4, 0.55) + generateTime(20.8, 0.55);
      |     dt = dt * 0.85
      |     elseif entity.Product == 20
      |     dt = generateTime (10.4, 0.55) + generateTime(25.1, 0.55);
      |     dt = dt * 0.85
      |     elseif entity.Product == 11
      |     dt = generateTime (12.1, 0.55) + generateTime (20.8, 0.55);
      |     dt = dt * 0.85
      |     elseif entity.Product == 21
      |     dt = generateTime (12.1, 0.55) + generateTime (25.1, 0.55);
      |     dt = dt * 0.85
      |     elseif entity.Product == 35
      |     dt = generateTime (12.1, 0.55) + generateTime (20.8, 0.55);
      |     dt = dt * 0.85
      |     else
      |     dt = 0;
      |     end
      | end
      | % Define persistent variables to track the total throughput time and entity count
      | persistent TTPtotal entityCount;
      | 
      | % Initialize the persistent variables if they are empty
      | if isempty(TTPtotal)
      |     TTPtotal = 0;
      | end
      | if isempty(entityCount)
      |     entityCount = 0;
      | end
      | 
      | % Read the current entity's final time and calculate throughput time
      | entity.EndTimeElec = ReadTime();
      | entity.TTPelec = abs(entity.EndTimeElec - entity.EndTimeHydTest);
      | 
      | % Update the total throughput time and entity count
      | TTPtotal = TTPtotal + entity.TTPelec;
      | entityCount = entityCount + 1;
      | 
      | % Calculate the average throughput time
      | avgTTPelec = TTPtotal / entityCount;
      | 
      | % Send the average throughput time to the workspace
      | ToWorkspace_ElecAssembly(avgTTPelec);
      settings: OutputPortMap=o5,o9
  Electronics Assembly with proposed upgrade Upgrade = Display mounting assist system DOUBLE UPGRADE extra capacity Process 9 and 10 : EntityServer  InputPortMessageModes=m  OutputPortMessageModes=n,m  Capacity=2  ServiceTimeSource=MATLAB action  ServiceTimeValue=32  ServiceTimeAction=|  ServiceCompleteAction=|  Utilization=on
      | generateTime = @(mu, cv) lognrnd(log(mu) - 0.5*log(1+cv^2), sqrt(log(1+cv^2)));
      | 
      | if entity.ElecReworked == 1
      |     dt = 1;
      | else
      |     if entity.Product == 1
      |     dt = generateTime(10.4, 0.55)  * 0.75+ generateTime(20.8, 0.55);
      |     elseif entity.Product == 3
      |     dt = generateTime (10.4, 0.55) * 0.75 + generateTime(25.1, 0.55);
      |     elseif entity.Product == 2
      |     dt = generateTime (12.1, 0.55) * 0.75 + generateTime (20.8, 0.55);
      |     elseif entity.Product == 4
      |     dt = generateTime (12.1, 0.55) * 0.75 + generateTime (25.1, 0.55);
      |     elseif entity.Product == 5
      |     dt = generateTime (12.1, 0.55) * 0.75 + generateTime (20.8, 0.55);
      |     else
      |     dt = 0;
      |     end
      | end
      | 
      | % Setup times
      | persistent last_product;
      | 
      | if isempty(last_product)
      |     last_product = 0;
      | end
      | 
      | setuptime = 0;
      | 
      | if last_product == 0
      |     % First entity - no setup time needed
      |     setuptime = 0;
      | elseif last_product ~= entity.Product
      |     % Product change detected - apply setup time based on previous product
      |     setuptime = 0.5;
      | end
      | 
      | dt = dt + setuptime;
      | last_product = entity.Product;
      | % Define persistent variables to track the total throughput time and entity count
      | persistent TTPtotal entityCount;
      | 
      | % Initialize the persistent variables if they are empty
      | if isempty(TTPtotal)
      |     TTPtotal = 0;
      | end
      | if isempty(entityCount)
      |     entityCount = 0;
      | end
      | 
      | % Read the current entity's final time and calculate throughput time
      | entity.EndTimeElec = ReadTime();
      | entity.TTPelec = abs(entity.EndTimeElec - entity.EndTimeHydTest);
      | 
      | % Update the total throughput time and entity count
      | TTPtotal = TTPtotal + entity.TTPelec;
      | entityCount = entityCount + 1;
      | 
      | % Calculate the average throughput time
      | avgTTPelec = TTPtotal / entityCount;
      | 
      | % Send the average throughput time to the workspace
      | ToWorkspace_ElecAssembly(avgTTPelec);
      settings: OutputPortMap=o5,o9
  Electronics Assembly with proposed upgrade Upgrade = extra workbench Process 9 and 10 Capacity = 1 : EntityServer  Commented=on  InputPortMessageModes=m  OutputPortMessageModes=n,m  Capacity=3  ServiceTimeSource=MATLAB action  ServiceTimeValue=32  ServiceTimeAction=|  ServiceCompleteAction=|  Utilization=on
      | generateTime = @(mu, cv) lognrnd(log(mu) - 0.5*log(1+cv^2), sqrt(log(1+cv^2)));
      | 
      | if entity.ElecReworked == 1
      |     dt = 1;
      | else
      |     if entity.Product == 10
      |     dt = generateTime(10.4, 0.55) + generateTime(20.8, 0.55);
      |     elseif entity.Product == 20
      |     dt = generateTime (10.4, 0.55) + generateTime(25.1, 0.55);
      |     elseif entity.Product == 11
      |     dt = generateTime (12.1, 0.55) + generateTime (20.8, 0.55);
      |     elseif entity.Product == 21
      |     dt = generateTime (12.1, 0.55) + generateTime (25.1, 0.55);
      |     elseif entity.Product == 35
      |     dt = generateTime (12.1, 0.55) + generateTime (20.8, 0.55);
      |     else
      |     dt = 0;
      |     end
      | end
      | % Define persistent variables to track the total throughput time and entity count
      | persistent TTPtotal entityCount;
      | 
      | % Initialize the persistent variables if they are empty
      | if isempty(TTPtotal)
      |     TTPtotal = 0;
      | end
      | if isempty(entityCount)
      |     entityCount = 0;
      | end
      | 
      | % Read the current entity's final time and calculate throughput time
      | entity.EndTimeElec = ReadTime();
      | entity.TTPelec = abs(entity.EndTimeElec - entity.EndTimeHydTest);
      | 
      | % Update the total throughput time and entity count
      | TTPtotal = TTPtotal + entity.TTPelec;
      | entityCount = entityCount + 1;
      | 
      | % Calculate the average throughput time
      | avgTTPelec = TTPtotal / entityCount;
      | 
      | % Send the average throughput time to the workspace
      | ToWorkspace_ElecAssembly(avgTTPelec);
      settings: OutputPortMap=o5,o9
  Electronics Testing Process 11 Capacity = 1 : EntityServer  Commented=on  InputPortMessageModes=m  OutputPortMessageModes=n,m  Capacity=1  ServiceTimeSource=MATLAB action  ServiceTimeValue=18  ServiceTimeAction=|  ServiceCompleteAction=|  SortingAttributeName=ElectronicsResult  ResidualTimeAttributeName=HydraulicsResult  Utilization=on
      | generateTime = @(mu, cv) lognrnd(log(mu) - 0.5*log(1+cv^2), sqrt(log(1+cv^2)));
      | 
      | if entity.Product == 1 | entity.Product == 2
      |     dt = generateTime (6.5, 0.4);
      | elseif entity.Product == 3 | entity.Product == 4 | entity.Product == 5
      |     dt = generateTime (10.4, 0.4);
      | else
      |     dt = 0;
      | end
      | 
      | if dt <= 0
      |     dt = 0;
      | end
      | 
      | % Setup times
      | persistent last_product;
      | 
      | if isempty(last_product)
      |     last_product = 0;
      | end
      | 
      | setuptime = 0;
      | 
      | if last_product == 0
      |     % First entity - no setup time needed
      |     setuptime = 0;
      | elseif last_product ~= entity.Product
      |     % Product change detected - apply setup time based on previous product
      |     setuptime = 0.5;
      | end
      | 
      | dt = dt + setuptime;
      | last_product = entity.Product;
      | % Define persistent variables to track the total throughput time and entity count
      | persistent TTPtotal entityCount;
      | 
      | % Initialize the persistent variables if they are empty
      | if isempty(TTPtotal)
      |     TTPtotal = 0;
      | end
      | if isempty(entityCount)
      |     entityCount = 0;
      | end
      | 
      | % Read the current entity's final time and calculate throughput time
      | entity.EndTimeElecTest = ReadTime();
      | entity.TTPelectest = abs(entity.EndTimeElecTest - entity.EndTimeElec);
      | 
      | % Update the total throughput time and entity count
      | TTPtotal = TTPtotal + entity.TTPelectest;
      | entityCount = entityCount + 1;
      | 
      | % Calculate the average throughput time
      | avgTTPelectest = TTPtotal / entityCount;
      | 
      | % Send the average throughput time to the workspace
      | ToWorkspace_ElecTest(avgTTPelectest);
      settings: OutputPortMap=o5,o9
  Electronics Testing with proposed upgrade Upgrade = Automated CPU burn-in testing Impact = Test time -20% Process 11 Capacity = 1 : EntityServer  InputPortMessageModes=m  OutputPortMessageModes=n,m  Capacity=1  ServiceTimeSource=MATLAB action  ServiceTimeValue=18  ServiceTimeAction=|  ServiceCompleteAction=|  SortingAttributeName=ElectronicsResult  ResidualTimeAttributeName=HydraulicsResult  Utilization=on
      | generateTime = @(mu, cv) lognrnd(log(mu) - 0.5*log(1+cv^2), sqrt(log(1+cv^2)));
      | 
      | if entity.Product == 1 | entity.Product == 2
      |     dt = generateTime (6.5, 0.4);
      |     dt = dt * 0.8;
      | elseif entity.Product == 3 | entity.Product == 4 | entity.Product == 5
      |     dt = generateTime (10.4, 0.4);
      |     dt = dt * 0.8;
      | else
      |     dt = 0;
      | end
      | 
      | if dt <= 0
      |     dt = 0;
      | end
      | 
      | % Setup times
      | persistent last_product;
      | last_product = 0;
      | setuptime = 0;
      | if last_product == 0
      |     last_product = entity.Product;   % first entity
      |     dt = dt + setuptime;
      | else
      |     if last_product == entity.Product;
      |         dt = dt + setuptime;
      |     else
      |         if last_product ~= entity.Product
      |             setuptime = 0.5;
      |             dt = dt + setuptime;
      |         end
      |     end
      |     last_product = entity.Product;
      | end
      | % Define persistent variables to track the total throughput time and entity count
      | persistent TTPtotal entityCount;
      | 
      | % Initialize the persistent variables if they are empty
      | if isempty(TTPtotal)
      |     TTPtotal = 0;
      | end
      | if isempty(entityCount)
      |     entityCount = 0;
      | end
      | 
      | % Read the current entity's final time and calculate throughput time
      | entity.EndTimeElecTest = ReadTime();
      | entity.TTPelectest = abs(entity.EndTimeElecTest - entity.EndTimeElec);
      | 
      | % Update the total throughput time and entity count
      | TTPtotal = TTPtotal + entity.TTPelectest;
      | entityCount = entityCount + 1;
      | 
      | % Calculate the average throughput time
      | avgTTPelectest = TTPtotal / entityCount;
      | 
      | % Send the average throughput time to the workspace
      | ToWorkspace_ElecTest(avgTTPelectest);
      settings: OutputPortMap=o5,o9
  Entity Input Switch : EntityInputSwitch  InputPortMessageModes=m,m  OutputPortMessageModes=m
  Entity Input Switch1 : EntityInputSwitch  InputPortMessageModes=m,m  OutputPortMessageModes=m
  Entity Input Switch2 : EntityInputSwitch  InputPortMessageModes=m,m  OutputPortMessageModes=m
  Entity Output Switch : EntityOutputSwitch  InputPortMessageModes=m  OutputPortMessageModes=m,m,m  NumberOutputPorts=3  SwitchingCriterion=From attribute  SwitchAttributeName=HydTestResult
      settings: OutputPortMap=o0,o1,o2
  Entity Output Switch1 : EntityOutputSwitch  InputPortMessageModes=m  OutputPortMessageModes=m,m,m  NumberOutputPorts=3  SwitchingCriterion=From attribute  SwitchAttributeName=ElecTestResult
      settings: OutputPortMap=o0,o1,o2
  Entity Output Switch2 : EntityOutputSwitch  InputPortMessageModes=m  OutputPortMessageModes=m,m,m  NumberOutputPorts=3  SwitchingCriterion=From attribute  SwitchAttributeName=FinalTestResult
      settings: OutputPortMap=o0,o1,o2
  Entity Output Switch3 : EntityOutputSwitch  InputPortMessageModes=m  OutputPortMessageModes=m,m,m,m,m  NumberOutputPorts=5  SwitchingCriterion=From attribute  SwitchAttributeName=Product
      settings: OutputPortMap=o0,o1,o2,o3,o4
  Entity Gate : EntityGate  InputPortMessageModes=m,m  OutputPortMessageModes=m
  Entity Gate1 : EntityGate  InputPortMessageModes=m,m  OutputPortMessageModes=m
  Entity Generator Proposed Solution on Boiler Assembly Reduces defects (rework and scrap) by 20% HAS TO BE PAIRED WITH ENTITY SERVER : EntityGenerator  OutputPortMessageModes=n,m  Period=16.09  GenerateAction=|  AttributeName=Product|HydTestResult|ElecTestResult|FinalTestResult|TimeInSystem|StartTime|EndTime|HydReworked|ElecReworked|FinalReworked|EndTimeChassis|EndTimeEbox|EndTimeBoiler|EndTimeValves|EndTimeHydTest|EndTimeElec|EndTimeElecTest|EndTimeComponents|EndTimeFinalTest|EndTimePainting|TTPchassis|TTPebox|TTPboiler|TTPvalves|TTPhydtest|TTPelec|TTPelectest|TTPcomponents|TTPfinaltest|TTPpainting|TTPpackaging  AttributeInitialValue=1|1|1|1|0|0|0|0|0|0|0|0|0|0|0|0|0|0|0|0|0|0|0|0|0|0|0|0|0|0|0  NumberEntitiesDeparted=on  EntityType=Structured  EntityTypeName=Entity
      | currentTime = ReadTime();
      | yearMinutes = 105600;
      | 
      | % Determine current year
      | if currentTime <= yearMinutes         % Year 1
      |     entity.Product = randsample([1, 2, 3, 4, 5], 1, true, ...
      |                                 [0.17, 0.15, 0.23, 0.26, 0.19]);
      |     
      |     
      | elseif currentTime <= 2*yearMinutes   % Year 3
      |     entity.Product = randsample([10, 20, 11, 21, 35], 1, true, ...
      |                                 [0.21, 0.19, 0.21, 0.24, 0.15]);
      | 
      | elseif currentTime <= 3*yearMinutes   % Year 4
      |     entity.Product = randsample([10, 20, 11, 21, 35], 1, true, ...
      |                                 [0.17, 0.15, 0.23, 0.26, 0.19]);
      | 
      | elseif currentTime <= 4*yearMinutes   % Year 5
      |     entity.Product = randsample([10, 20, 11, 21, 35], 1, true, ...
      |                                 [0.14, 0.12, 0.24, 0.28, 0.22]);
      | 
      | else   % Year 6
      |     entity.Product = randsample([10, 20, 11, 21, 35], 1, true, ...
      |                                 [0.11, 0.10, 0.25, 0.30, 0.24]);
      | end
      | 
      | % Assign testing results
      | entity.HydTestResult = randsample([1, 2, 3], 1, true, [0.912, 0.064, 0.024]);
      | entity.ElecTestResult = randsample([1, 2, 3], 1, true, [0.94, 0.06, 0]);
      | entity.FinalTestResult = randsample([1, 2, 3], 1, true, [0.87, 0.10, 0.03]);
      | 
      | % Track entry time
      | entity.StartTime = ReadTime();
      settings: OutputPortMap=o0,o3
  Entity Generator Proposed Solution on Chassis Assembly Reduces quality defects by 20% HAS TO BE PAIRED WITH ENTITY SERVER : EntityGenerator  Commented=on  OutputPortMessageModes=n,m  Period=18.5  GenerateAction=|  AttributeName=Product|HydTestResult|ElecTestResult|FinalTestResult|TimeInSystem|StartTime|EndTime|HydReworked|ElecReworked|FinalReworked|EndTimeChassis|EndTimeEbox|EndTimeBoiler|EndTimeValves|EndTimeHydTest|EndTimeElec|EndTimeElecTest|EndTimeComponents|EndTimeFinalTest|EndTimePainting|TTPchassis|TTPebox|TTPboiler|TTPvalves|TTPhydtest|TTPelec|TTPelectest|TTPcomponents|TTPfinaltest|TTPpainting|TTPpackaging  AttributeInitialValue=10|1|1|1|0|0|0|0|0|0|0|0|0|0|0|0|0|0|0|0|0|0|0|0|0|0|0|0|0|0|0  NumberEntitiesDeparted=on  EntityType=Structured  EntityTypeName=Entity
      | currentTime = ReadTime();
      | yearMinutes = 105600;
      | 
      | % Determine current year
      | if currentTime <= yearMinutes         % Year 1
      |     entity.Product = randsample([10, 20, 11, 21], 1, true, ...
      |                                 [0.37, 0.32, 0.14, 0.17]);
      | 
      | elseif currentTime <= 2*yearMinutes   % Year 2
      |     entity.Product = randsample([10, 20, 11, 21, 35], 1, true, ...
      |                                 [0.28, 0.24, 0.18, 0.22, 0.08]);
      | 
      | elseif currentTime <= 3*yearMinutes   % Year 3
      |     entity.Product = randsample([10, 20, 11, 21, 35], 1, true, ...
      |                                 [0.21, 0.19, 0.21, 0.24, 0.15]);
      | 
      | elseif currentTime <= 4*yearMinutes   % Year 4
      |     entity.Product = randsample([10, 20, 11, 21, 35], 1, true, ...
      |                                 [0.17, 0.15, 0.23, 0.26, 0.19]);
      | 
      | elseif currentTime <= 5*yearMinutes   % Year 5
      |     entity.Product = randsample([10, 20, 11, 21, 35], 1, true, ...
      |                                 [0.14, 0.12, 0.24, 0.28, 0.22]);
      | 
      | else   % Year 6
      |     entity.Product = randsample([10, 20, 11, 21, 35], 1, true, ...
      |                                 [0.11, 0.10, 0.25, 0.30, 0.24]);
      | end
      | 
      | % Assign testing results
      | entity.HydTestResult = randsample([1, 2, 3], 1, true, [0.9, 0.072, 0.024]);
      | entity.ElecTestResult = randsample([1, 2, 3], 1, true, [0.94, 0.06, 0]);
      | entity.FinalTestResult = randsample([1, 2, 3], 1, true, [0.87, 0.10, 0.03]);
      | 
      | % Track entry time
      | entity.StartTime = ReadTime();
      settings: OutputPortMap=o0,o3
  Entity Generator Proposed Solution on Components Assembly Reduces scrap and rework on final testing : EntityGenerator  Commented=on  OutputPortMessageModes=n,m  Period=18.5  GenerateAction=|  AttributeName=Product|HydTestResult|ElecTestResult|FinalTestResult|TimeInSystem|StartTime|EndTime|HydReworked|ElecReworked|FinalReworked|EndTimeChassis|EndTimeEbox|EndTimeBoiler|EndTimeValves|EndTimeHydTest|EndTimeElec|EndTimeElecTest|EndTimeComponents|EndTimeFinalTest|EndTimePainting|TTPchassis|TTPebox|TTPboiler|TTPvalves|TTPhydtest|TTPelec|TTPelectest|TTPcomponents|TTPfinaltest|TTPpainting|TTPpackaging  AttributeInitialValue=10|1|1|1|0|0|0|0|0|0|0|0|0|0|0|0|0|0|0|0|0|0|0|0|0|0|0|0|0|0|0  NumberEntitiesDeparted=on  EntityType=Structured  EntityTypeName=Entity
      | currentTime = ReadTime();
      | yearMinutes = 105600;
      | 
      | % Determine current year
      | if currentTime <= yearMinutes         % Year 1
      |     entity.Product = randsample([10, 20, 11, 21], 1, true, ...
      |                                 [0.37, 0.32, 0.14, 0.17]);
      | 
      | elseif currentTime <= 2*yearMinutes   % Year 2
      |     entity.Product = randsample([10, 20, 11, 21, 35], 1, true, ...
      |                                 [0.28, 0.24, 0.18, 0.22, 0.08]);
      | 
      | elseif currentTime <= 3*yearMinutes   % Year 3
      |     entity.Product = randsample([10, 20, 11, 21, 35], 1, true, ...
      |                                 [0.21, 0.19, 0.21, 0.24, 0.15]);
      | 
      | elseif currentTime <= 4*yearMinutes   % Year 4
      |     entity.Product = randsample([10, 20, 11, 21, 35], 1, true, ...
      |                                 [0.17, 0.15, 0.23, 0.26, 0.19]);
      | 
      | elseif currentTime <= 5*yearMinutes   % Year 5
      |     entity.Product = randsample([10, 20, 11, 21, 35], 1, true, ...
      |                                 [0.14, 0.12, 0.24, 0.28, 0.22]);
      | 
      | else   % Year 6
      |     entity.Product = randsample([10, 20, 11, 21, 35], 1, true, ...
      |                                 [0.11, 0.10, 0.25, 0.30, 0.24]);
      | end
      | 
      | % Assign testing results
      | entity.HydTestResult = randsample([1, 2, 3], 1, true, [0.89, 0.08, 0.03]);
      | entity.ElecTestResult = randsample([1, 2, 3], 1, true, [0.94, 0.06, 0]);
      | entity.FinalTestResult = randsample([1, 2, 3], 1, true, [0.94, 0.04, 0.02]);
      | 
      | % Track entry time
      | entity.StartTime = ReadTime();
      settings: OutputPortMap=o0,o3
  Entity Generator Proposed Solution on Electronic Assembly Reduces rework rate by 45% HAS TO BE PAIRED WITH ENTITY SERVER1 : EntityGenerator  Commented=on  OutputPortMessageModes=n,m  Period=18.5  GenerateAction=|  AttributeName=Product|HydTestResult|ElecTestResult|FinalTestResult|TimeInSystem|StartTime|EndTime|HydReworked|ElecReworked|FinalReworked|EndTimeChassis|EndTimeEbox|EndTimeBoiler|EndTimeValves|EndTimeHydTest|EndTimeElec|EndTimeElecTest|EndTimeComponents|EndTimeFinalTest|EndTimePainting|TTPchassis|TTPebox|TTPboiler|TTPvalves|TTPhydtest|TTPelec|TTPelectest|TTPcomponents|TTPfinaltest|TTPpainting|TTPpackaging  AttributeInitialValue=10|1|1|1|0|0|0|0|0|0|0|0|0|0|0|0|0|0|0|0|0|0|0|0|0|0|0|0|0|0|0  NumberEntitiesDeparted=on  EntityType=Structured  EntityTypeName=Entity
      | currentTime = ReadTime();
      | yearMinutes = 105600;
      | 
      | % Determine current year
      | if currentTime <= yearMinutes         % Year 1
      |     entity.Product = randsample([10, 20, 11, 21], 1, true, ...
      |                                 [0.37, 0.32, 0.14, 0.17]);
      | 
      | elseif currentTime <= 2*yearMinutes   % Year 2
      |     entity.Product = randsample([10, 20, 11, 21, 35], 1, true, ...
      |                                 [0.28, 0.24, 0.18, 0.22, 0.08]);
      | 
      | elseif currentTime <= 3*yearMinutes   % Year 3
      |     entity.Product = randsample([10, 20, 11, 21, 35], 1, true, ...
      |                                 [0.21, 0.19, 0.21, 0.24, 0.15]);
      | 
      | elseif currentTime <= 4*yearMinutes   % Year 4
      |     entity.Product = randsample([10, 20, 11, 21, 35], 1, true, ...
      |                                 [0.17, 0.15, 0.23, 0.26, 0.19]);
      | 
      | elseif currentTime <= 5*yearMinutes   % Year 5
      |     entity.Product = randsample([10, 20, 11, 21, 35], 1, true, ...
      |                                 [0.14, 0.12, 0.24, 0.28, 0.22]);
      | 
      | else   % Year 6
      |     entity.Product = randsample([10, 20, 11, 21, 35], 1, true, ...
      |                                 [0.11, 0.10, 0.25, 0.30, 0.24]);
      | end
      | 
      | % Assign testing results
      | entity.HydTestResult = randsample([1, 2, 3], 1, true, [0.912, 0.064, 0.024]);
      | entity.ElecTestResult = randsample([1, 2, 3], 1, true, [0.967, 0.033, 0]);
      | entity.FinalTestResult = randsample([1, 2, 3], 1, true, [0.87, 0.10, 0.03]);
      | 
      | % Track entry time
      | entity.StartTime = ReadTime();
      settings: OutputPortMap=o0,o3
  Entity Generator Proposed Solution on Electronics Assembly Reduces scrap and rework on electronics testing : EntityGenerator  Commented=on  OutputPortMessageModes=n,m  Period=18.5  GenerateAction=|  AttributeName=Product|HydTestResult|ElecTestResult|FinalTestResult|TimeInSystem|StartTime|EndTime|HydReworked|ElecReworked|FinalReworked|EndTimeChassis|EndTimeEbox|EndTimeBoiler|EndTimeValves|EndTimeHydTest|EndTimeElec|EndTimeElecTest|EndTimeComponents|EndTimeFinalTest|EndTimePainting|TTPchassis|TTPebox|TTPboiler|TTPvalves|TTPhydtest|TTPelec|TTPelectest|TTPcomponents|TTPfinaltest|TTPpainting|TTPpackaging  AttributeInitialValue=10|1|1|1|0|0|0|0|0|0|0|0|0|0|0|0|0|0|0|0|0|0|0|0|0|0|0|0|0|0|0  NumberEntitiesDeparted=on  EntityType=Structured  EntityTypeName=Entity
      | currentTime = ReadTime();
      | yearMinutes = 105600;
      | 
      | % Determine current year
      | if currentTime <= yearMinutes         % Year 1
      |     entity.Product = randsample([10, 20, 11, 21], 1, true, ...
      |                                 [0.37, 0.32, 0.14, 0.17]);
      | 
      | elseif currentTime <= 2*yearMinutes   % Year 2
      |     entity.Product = randsample([10, 20, 11, 21, 35], 1, true, ...
      |                                 [0.28, 0.24, 0.18, 0.22, 0.08]);
      | 
      | elseif currentTime <= 3*yearMinutes   % Year 3
      |     entity.Product = randsample([10, 20, 11, 21, 35], 1, true, ...
      |                                 [0.21, 0.19, 0.21, 0.24, 0.15]);
      | 
      | elseif currentTime <= 4*yearMinutes   % Year 4
      |     entity.Product = randsample([10, 20, 11, 21, 35], 1, true, ...
      |                                 [0.17, 0.15, 0.23, 0.26, 0.19]);
      | 
      | elseif currentTime <= 5*yearMinutes   % Year 5
      |     entity.Product = randsample([10, 20, 11, 21, 35], 1, true, ...
      |                                 [0.14, 0.12, 0.24, 0.28, 0.22]);
      | 
      | else   % Year 6
      |     entity.Product = randsample([10, 20, 11, 21, 35], 1, true, ...
      |                                 [0.11, 0.10, 0.25, 0.30, 0.24]);
      | end
      | 
      | % Assign testing results
      | entity.HydTestResult = randsample([1, 2, 3], 1, true, [0.89, 0.08, 0.03]);
      | entity.ElecTestResult = randsample([1, 2, 3], 1, true, [0.976, 0.024, 0]);
      | entity.FinalTestResult = randsample([1, 2, 3], 1, true, [0.87, 0.10, 0.03]);
      | 
      | % Track entry time
      | entity.StartTime = ReadTime();
      settings: OutputPortMap=o0,o3
  Entity Queue : Queue  InputPortMessageModes=m  OutputPortMessageModes=n,n,n,m  Capacity=inf  NumberEntitiesDeparted=on  NumberEntitiesInBlock=on  AverageWait=on
      settings: OutputPortMap=o0,o1,o2,o5
  Entity Queue1 : Queue  InputPortMessageModes=m  OutputPortMessageModes=n,n,n,m  Capacity=inf  QueueType=Priority  PrioritySource=HydReworked  SortingDirection=Descending  NumberEntitiesDeparted=on  NumberEntitiesInBlock=on  AverageWait=on
      settings: OutputPortMap=o0,o1,o2,o5
  Entity Queue10 : Queue  InputPortMessageModes=m  OutputPortMessageModes=n,n,n,m  Capacity=inf  PrioritySource=ReworkMachine  SortingDirection=Descending  NumberEntitiesDeparted=on  NumberEntitiesInBlock=on  AverageWait=on
      settings: OutputPortMap=o0,o1,o2,o5
  Entity Queue11 : Queue  InputPortMessageModes=m  OutputPortMessageModes=m  Capacity=inf
  Entity Queue12 : Queue  InputPortMessageModes=m  OutputPortMessageModes=m  Capacity=inf
  Entity Queue13 : Queue  InputPortMessageModes=m  OutputPortMessageModes=m  Capacity=inf
  Entity Queue2 : Queue  InputPortMessageModes=m  OutputPortMessageModes=n,n,n,m  Capacity=inf  QueueType=Priority  PrioritySource=HydReworked  SortingDirection=Descending  NumberEntitiesDeparted=on  NumberEntitiesInBlock=on  AverageWait=on
      settings: OutputPortMap=o0,o1,o2,o5
  Entity Queue3 : Queue  InputPortMessageModes=m  OutputPortMessageModes=n,n,n,m  NumberEntitiesDeparted=on  NumberEntitiesInBlock=on  AverageWait=on
      settings: OutputPortMap=o0,o1,o2,o5
  Entity Queue4 : Queue  InputPortMessageModes=m  OutputPortMessageModes=n,n,n,m  QueueType=Priority  PrioritySource=ElecReworked  NumberEntitiesDeparted=on  NumberEntitiesInBlock=on  AverageWait=on
      settings: OutputPortMap=o0,o1,o2,o5
  Entity Queue5 : Queue  InputPortMessageModes=m  OutputPortMessageModes=n,n,n,m  NumberEntitiesDeparted=on  NumberEntitiesInBlock=on  AverageWait=on
      settings: OutputPortMap=o0,o1,o2,o5
  Entity Queue6 : Queue  InputPortMessageModes=m  OutputPortMessageModes=n,n,n,m  Capacity=inf  PrioritySource=ReworkMachine  SortingDirection=Descending  NumberEntitiesDeparted=on  NumberEntitiesInBlock=on  AverageWait=on
      settings: OutputPortMap=o0,o1,o2,o5
  Entity Queue7 : Queue  InputPortMessageModes=m  OutputPortMessageModes=n,n,n,m  Capacity=inf  QueueType=Priority  PrioritySource=FinalReworked  SortingDirection=Descending  NumberEntitiesDeparted=on  NumberEntitiesInBlock=on  AverageWait=on
      settings: OutputPortMap=o0,o1,o2,o5
  Entity Queue8 : Queue  InputPortMessageModes=m  OutputPortMessageModes=n,n,n,m  Capacity=inf  NumberEntitiesDeparted=on  NumberEntitiesInBlock=on  AverageWait=on
      settings: OutputPortMap=o0,o1,o2,o5
  Entity Queue9 : Queue  InputPortMessageModes=m  OutputPortMessageModes=n,n,n,m  Capacity=inf  NumberEntitiesDeparted=on  NumberEntitiesInBlock=on  AverageWait=on
      settings: OutputPortMap=o0,o1,o2,o5
  Entity Replicator : EntityReplicator  InputPortMessageModes=m  OutputPortMessageModes=m,m  ReplicasDepartFrom=Single output port  NumberReplicas=30  HoldOriginalEntityUntilAllReplicasDepart=on
  Entity Server : EntityServer  InputPortMessageModes=m  OutputPortMessageModes=n,m  Capacity=1  ServiceTimeValue=0  EntryAction=|  NumberEntitiesDeparted=on
      | entity.HydTestResult = 1;
      | entity.HydReworked = 1;
      settings: OutputPortMap=o0,o9
  Entity Server1 : EntityServer  InputPortMessageModes=m  OutputPortMessageModes=n,m  Capacity=1  ServiceTimeValue=0  EntryAction=|  NumberEntitiesDeparted=on
      | entity.ElecTestResult = 1;
      | entity.ElecReworked = 1;
      settings: OutputPortMap=o0,o9
  Entity Server2 : EntityServer  InputPortMessageModes=m  OutputPortMessageModes=n,m  Capacity=1  ServiceTimeValue=0  EntryAction=|  NumberEntitiesDeparted=on
      | entity.FinalTestResult = 1;
      | entity.FinalReworked = 1;
      settings: OutputPortMap=o0,o9
  Entity Terminator : EntityTerminator  InputPortMessageModes=m  NumberEntitiesArrived=on
      settings: OutputPortMap=o0
  Entity Terminator1 : EntityTerminator  InputPortMessageModes=m  NumberEntitiesArrived=on
      settings: OutputPortMap=o0
  Entity Terminator2 : EntityTerminator  InputPortMessageModes=m  NumberEntitiesArrived=on
      settings: OutputPortMap=o0
  Entity Terminator3 : EntityTerminator  InputPortMessageModes=m  EntryAction=|  NumberEntitiesArrived=on
      | entity.EndTime = ReadTime();
      | entity.TimeInSystem = abs(entity.EndTime - entity.StartTime);
      | Workspace_Product_TimeInSystem(entity.Product, entity.TimeInSystem);
      settings: OutputPortMap=o0
  Entity Terminator4 : EntityTerminator  InputPortMessageModes=m  EntryAction=|  NumberEntitiesArrived=on
      | entity.EndTime = ReadTime();
      | entity.TimeInSystem = abs(entity.EndTime - entity.StartTime);
      | Workspace_Product_TimeInSystem(entity.Product, entity.TimeInSystem);
      settings: OutputPortMap=o0
  Entity Terminator5 : EntityTerminator  InputPortMessageModes=m  EntryAction=|  NumberEntitiesArrived=on
      | entity.EndTime = ReadTime();
      | entity.TimeInSystem = abs(entity.EndTime - entity.StartTime);
      | Workspace_Product_TimeInSystem(entity.Product, entity.TimeInSystem);
      settings: OutputPortMap=o0
  Entity Terminator6 : EntityTerminator  InputPortMessageModes=m  EntryAction=|  NumberEntitiesArrived=on
      | entity.EndTime = ReadTime();
      | entity.TimeInSystem = abs(entity.EndTime - entity.StartTime);
      | Workspace_Product_TimeInSystem(entity.Product, entity.TimeInSystem);
      settings: OutputPortMap=o0
  Entity Terminator7 : EntityTerminator  InputPortMessageModes=m  EntryAction=|  NumberEntitiesArrived=on
      | entity.EndTime = ReadTime();
      | entity.TimeInSystem = abs(entity.EndTime - entity.StartTime);
      | Workspace_Product_TimeInSystem(entity.Product, entity.TimeInSystem);
      settings: OutputPortMap=o0
  Entity Terminator8 : EntityTerminator  InputPortMessageModes=m
  Final Testing Process 14 Capacity = 1 : EntityServer  Commented=on  InputPortMessageModes=m  OutputPortMessageModes=n,m  Capacity=2  ServiceTimeSource=MATLAB action  ServiceTimeValue=32  ServiceTimeAction=|  ServiceCompleteAction=|  Utilization=on
      ServiceTimeAction=|
      | % Assign testing times based on product code
      | 
      | if entity.Product == 1 | entity.Product == 2
      |     dt = 18.2;
      | elseif entity.Product == 3 | entity.Product == 4
      |     dt = 13;
      | elseif entity.Product == 5
      |     dt = 20.8;
      | else
      |     dt = 0; 
      | end
      | 
      | % Setup times
      | persistent last_product;
      | 
      | if isempty(last_product)
      |     last_product = 0;
      | end
      | 
      | setuptime = 0;
      | 
      | if last_product == 0
      |     % First entity - no setup time needed
      |     setuptime = 0;
      | elseif last_product ~= entity.Product
      |     % Product change detected - apply setup time based on previous product
      |     setuptime = 0.5;
      | end
      | 
      | dt = dt + setuptime;
      | last_product = entity.Product;
      ServiceCompleteAction=|
      | % Define persistent variables to track the total throughput time and entity count
      | persistent TTPtotal entityCount;
      | 
      | % Initialize the persistent variables if they are empty
      | if isempty(TTPtotal)
      |     TTPtotal = 0;
      | end
      | if isempty(entityCount)
      |     entityCount = 0;
      | end
      | 
      | % Read the current entity's final time and calculate throughput time
      | entity.EndTimeFinalTest = ReadTime();
      | entity.TTPfinaltest = abs(entity.EndTimeFinalTest - entity.EndTimeComponents);
      | 
      | % Update the total throughput time and entity count
      | TTPtotal = TTPtotal + entity.TTPfinaltest;
      | entityCount = entityCount + 1;
      | 
      | % Calculate the average throughput time
      | avgTTPfinaltest = TTPtotal / entityCount;
      | 
      | % Send the average throughput time to the workspace
      | ToWorkspace_FinalTest(avgTTPfinaltest);
      settings: OutputPortMap=o5,o9
  Final testing with proposed upgrade Upgrade = AI optimized testing routines DOUBLE UPGRADE enhanced station Process 14 Capacity = 2 : EntityServer  InputPortMessageModes=m  OutputPortMessageModes=n,m  Capacity=2  ServiceTimeSource=MATLAB action  ServiceTimeValue=32  ServiceTimeAction=|  ServiceCompleteAction=|  Utilization=on
      ServiceTimeAction=|
      | % Assign testing times based on product code
      | 
      | if entity.Product == 1 | entity.Product == 3
      |     dt = 18.2 * 0.8;
      | elseif entity.Product == 2 | entity.Product == 4
      |     dt = 13 * 0.8;
      | elseif entity.Product == 35
      |     dt = 20.8 * 0.8;
      | else
      |     dt = 0; 
      | end
      | 
      | dt = dt * 0.8;
      | 
      | % Setup times
      | persistent last_product;
      | 
      | if isempty(last_product)
      |     last_product = 0;
      | end
      | 
      | setuptime = 0;
      | 
      | if last_product == 0
      |     % First entity - no setup time needed
      |     setuptime = 0;
      | elseif last_product ~= entity.Product
      |     % Product change detected - apply setup time based on previous product
      |     setuptime = 0.5;
      | end
      | 
      | dt = dt + setuptime;
      | last_product = entity.Product;
      ServiceCompleteAction=|
      | % Define persistent variables to track the total throughput time and entity count
      | persistent TTPtotal entityCount;
      | 
      | % Initialize the persistent variables if they are empty
      | if isempty(TTPtotal)
      |     TTPtotal = 0;
      | end
      | if isempty(entityCount)
      |     entityCount = 0;
      | end
      | 
      | % Read the current entity's final time and calculate throughput time
      | entity.EndTimeFinalTest = ReadTime();
      | entity.TTPfinaltest = abs(entity.EndTimeFinalTest - entity.EndTimeComponents);
      | 
      | % Update the total throughput time and entity count
      | TTPtotal = TTPtotal + entity.TTPfinaltest;
      | entityCount = entityCount + 1;
      | 
      | % Calculate the average throughput time
      | avgTTPfinaltest = TTPtotal / entityCount;
      | 
      | % Send the average throughput time to the workspace
      | ToWorkspace_FinalTest(avgTTPfinaltest);
      settings: OutputPortMap=o5,o9
  Final testing with proposed upgrade Upgrade = Enhanced machine testing station Process 14 Capacity = 1 : EntityServer  Commented=on  InputPortMessageModes=m  OutputPortMessageModes=n,m  Capacity=2  ServiceTimeSource=MATLAB action  ServiceTimeValue=32  ServiceTimeAction=|  ServiceCompleteAction=|  Utilization=on
      ServiceTimeAction=|
      | % Assign testing times based on product code
      | 
      | if entity.Product == 10 | entity.Product == 20
      |     dt = 18.2 * 0.8;
      | elseif entity.Product == 11 | entity.Product == 21
      |     dt = 13 * 0.8;
      | elseif entity.Product == 35
      |     dt = 20.8 * 0.8;
      | else
      |     dt = 0; 
      | end
      ServiceCompleteAction=|
      | % Define persistent variables to track the total throughput time and entity count
      | persistent TTPtotal entityCount;
      | 
      | % Initialize the persistent variables if they are empty
      | if isempty(TTPtotal)
      |     TTPtotal = 0;
      | end
      | if isempty(entityCount)
      |     entityCount = 0;
      | end
      | 
      | % Read the current entity's final time and calculate throughput time
      | entity.EndTimeFinalTest = ReadTime();
      | entity.TTPfinaltest = abs(entity.EndTimeFinalTest - entity.EndTimeComponents);
      | 
      | % Update the total throughput time and entity count
      | TTPtotal = TTPtotal + entity.TTPfinaltest;
      | entityCount = entityCount + 1;
      | 
      | % Calculate the average throughput time
      | avgTTPfinaltest = TTPtotal / entityCount;
      | 
      | % Send the average throughput time to the workspace
      | ToWorkspace_FinalTest(avgTTPfinaltest);
      settings: OutputPortMap=o5,o9
  From Workspace : FromWorkspace  VariableName=MTBF_MTTR_EBOX_smartsensors
  From Workspace1 : FromWorkspace  VariableName=MTBF_MTTR_PAINT_predictive
  Gain{,1..8} (9 alike) : Gain
  Hydraulics Testing Process 8 Capacity = 1 : EntityServer  Commented=on  InputPortMessageModes=m  OutputPortMessageModes=n,m  Capacity=1  ServiceTimeSource=MATLAB action  ServiceTimeValue=18  ServiceTimeAction=|  ServiceCompleteAction=|  SortingAttributeName=HydReworked  Utilization=on
      ServiceTimeAction=|
      | % The service time is the same for all product types
      | % Process time
      | dt = 18;
      | 
      | % Setup times
      | persistent last_product;
      | 
      | if isempty(last_product)
      |     last_product = 0;
      | end
      | 
      | setuptime = 0;
      | 
      | if last_product == 0
      |     % First entity - no setup time needed
      |     setuptime = 0;
      | elseif last_product ~= entity.Product
      |     % Product change detected - apply setup time based on previous product
      |     setuptime = 4;
      | end
      | 
      | dt = dt + setuptime;
      | last_product = entity.Product;
      ServiceCompleteAction=|
      | % Define persistent variables to track the total throughput time and entity count
      | persistent TTPtotal entityCount;
      | % TTPtotal = tracks the total TTP of the system. In which, when every new station is visited, the time is added
      | % entityCount =
      | 
      | % Initialize the persistent variables if they are empty
      | if isempty(TTPtotal)
      |     TTPtotal = 0;
      | end
      | if isempty(entityCount)
      |     entityCount = 0;
      | end
      | 
      | % Read the current entity's final time
      | entity.EndTimeHydTest = ReadTime();
      | 
      | % Calculate the TTP for the chassis department for the specific entity
      | % INCLUDES wait time
      | entity.TTPhydtest = abs(entity.EndTimeHydTest - entity.EndTimeValves);
      | 
      | % Update the total throughput time and entity count
      | % This is done AFTER the process, 
      |     % to mark that the entity has gone through the chassis department 
      |         % (thus TTPchassis being added)
      |             % and add that the entity, for each entity after being processed
      |             
      | TTPtotal = TTPtotal + entity.TTPhydtest;
      | entityCount = entityCount + 1;
      | 
      | % Calculate the average throughput time for the chassis department
      | avgTTPhydtest = TTPtotal / entityCount;
      | 
      | % Send the average throughput time to the workspace
      | ToWorkspace_HydTest(avgTTPhydtest);
      settings: OutputPortMap=o5,o9
  Hydraulics Testing with proposed upgrade Upgrade = AI optimized testing routines Process 8 Capacity = 1 : EntityServer  Commented=on  InputPortMessageModes=m  OutputPortMessageModes=n,m  Capacity=1  ServiceTimeValue=14.4  ServiceTimeAction=|  ServiceCompleteAction=|  SortingAttributeName=HydReworked  Utilization=on
      ServiceTimeAction=|
      | % It is easier to use dialog
      | % But i just want to demonstrate that
      | % The service time is the same for all product types
      | 
      | dt = 32
      ServiceCompleteAction=|
      | % Define persistent variables to track the total throughput time and entity count
      | persistent TTPtotal entityCount;
      | % TTPtotal = tracks the total TTP of the system. In which, when every new station is visited, the time is added
      | % entityCount =
      | 
      | % Initialize the persistent variables if they are empty
      | if isempty(TTPtotal)
      |     TTPtotal = 0;
      | end
      | if isempty(entityCount)
      |     entityCount = 0;
      | end
      | 
      | % Read the current entity's final time
      | entity.EndTimeHydTest = ReadTime();
      | 
      | % Calculate the TTP for the chassis department for the specific entity
      | % INCLUDES wait time
      | entity.TTPhydtest = abs(entity.EndTimeHydTest - entity.EndTimeValves);
      | 
      | % Update the total throughput time and entity count
      | % This is done AFTER the process, 
      |     % to mark that the entity has gone through the chassis department 
      |         % (thus TTPchassis being added)
      |             % and add that the entity, for each entity after being processed
      |             
      | TTPtotal = TTPtotal + entity.TTPhydtest;
      | entityCount = entityCount + 1;
      | 
      | % Calculate the average throughput time for the chassis department
      | avgTTPhydtest = TTPtotal / entityCount;
      | 
      | % Send the average throughput time to the workspace
      | ToWorkspace_HydTest(avgTTPhydtest);
      settings: OutputPortMap=o5,o9
  Hydraulics Testing with proposed upgrade Upgrade = Automated parallel multimachine hyd testing cell DOUBLE upgrade AI optimized testing routines Process 8 Capacity = 2 : EntityServer  InputPortMessageModes=m  OutputPortMessageModes=n,m  Capacity=2  ServiceTimeSource=MATLAB action  ServiceTimeValue=9  ServiceTimeAction=|  ServiceCompleteAction=|  SortingAttributeName=HydReworked  Utilization=on
      ServiceTimeAction=|
      | dt = 9;
      | 
      | 
      | % Setup times
      | persistent last_product;
      | 
      | if isempty(last_product)
      |     last_product = 0;
      | end
      | 
      | setuptime = 0;
      | 
      | if last_product == 0
      |     % First entity - no setup time needed
      |     setuptime = 0;
      | elseif last_product ~= entity.Product
      |     % Product change detected - apply setup time based on previous product
      |     setuptime = 4;
      | end
      | 
      | dt = dt + setuptime;
      | last_product = entity.Product;
      ServiceCompleteAction=|
      | % Define persistent variables to track the total throughput time and entity count
      | persistent TTPtotal entityCount;
      | % TTPtotal = tracks the total TTP of the system. In which, when every new station is visited, the time is added
      | % entityCount =
      | 
      | % Initialize the persistent variables if they are empty
      | if isempty(TTPtotal)
      |     TTPtotal = 0;
      | end
      | if isempty(entityCount)
      |     entityCount = 0;
      | end
      | 
      | % Read the current entity's final time
      | entity.EndTimeHydTest = ReadTime();
      | 
      | % Calculate the TTP for the chassis department for the specific entity
      | % INCLUDES wait time
      | entity.TTPhydtest = abs(entity.EndTimeHydTest - entity.EndTimeValves);
      | 
      | % Update the total throughput time and entity count
      | % This is done AFTER the process, 
      |     % to mark that the entity has gone through the chassis department 
      |         % (thus TTPchassis being added)
      |             % and add that the entity, for each entity after being processed
      |             
      | TTPtotal = TTPtotal + entity.TTPhydtest;
      | entityCount = entityCount + 1;
      | 
      | % Calculate the average throughput time for the chassis department
      | avgTTPhydtest = TTPtotal / entityCount;
      | 
      | % Send the average throughput time to the workspace
      | ToWorkspace_HydTest(avgTTPhydtest);
      settings: OutputPortMap=o5,o9
  Packaging Process 16 Capacity = 1 : EntityServer  Commented=on  InputPortMessageModes=m  OutputPortMessageModes=n,m  Capacity=1  ServiceTimeSource=MATLAB action  ServiceTimeValue=32  ServiceTimeAction=|  ServiceCompleteAction=|  Utilization=on
      | generateTime = @(mu, cv) lognrnd(log(mu) - 0.5*log(1+cv^2), sqrt(log(1+cv^2)));
      | 
      | dt = generateTime (18.2, 0.65);
      | if dt <= 0
      |     dt = 0;
      | end
      | 
      | % Setup times
      | persistent last_product;
      | 
      | if isempty(last_product)
      |     last_product = 0;
      | end
      | 
      | setuptime = 0;
      | 
      | if last_product == 0
      |     % First entity - no setup time needed
      |     setuptime = 0;
      | elseif last_product ~= entity.Product
      |     % Product change detected - apply setup time based on previous product
      |     setuptime = 1;
      | end
      | 
      | dt = dt + setuptime;
      | last_product = entity.Product;
      | % Define persistent variables to track the total throughput time and entity count
      | persistent TTPtotal entityCount;
      | 
      | % Initialize the persistent variables if they are empty
      | if isempty(TTPtotal)
      |     TTPtotal = 0;
      | end
      | if isempty(entityCount)
      |     entityCount = 0;
      | end
      | 
      | % Read the current entity's final time and calculate throughput time
      | entity.EndTime = ReadTime();
      | entity.TTPpackaging = abs(entity.EndTime - entity.EndTimePainting);
      | 
      | % Update the total throughput time and entity count
      | TTPtotal = TTPtotal + entity.TTPpackaging;
      | entityCount = entityCount + 1;
      | 
      | % Calculate the average throughput time
      | avgTTPpackaging = TTPtotal / entityCount;
      | 
      | % Send the average throughput time to the workspace
      | ToWorkspace_Packaging(avgTTPpackaging);
      settings: OutputPortMap=o5,o9
  Packaging Process 16 Capacity = Upgraded : EntityServer  Commented=on  InputPortMessageModes=m  OutputPortMessageModes=n,m  Capacity=2  ServiceTimeSource=MATLAB action  ServiceTimeValue=32  ServiceTimeAction=|  ServiceCompleteAction=|  Utilization=on
      | generateTime = @(mu, cv) lognrnd(log(mu) - 0.5*log(1+cv^2), sqrt(log(1+cv^2)));
      | 
      | dt = generateTime (18.2, 0.65);
      | if dt <= 0
      |     dt = 0;
      | end
      | % Define persistent variables to track the total throughput time and entity count
      | persistent TTPtotal entityCount;
      | 
      | % Initialize the persistent variables if they are empty
      | if isempty(TTPtotal)
      |     TTPtotal = 0;
      | end
      | if isempty(entityCount)
      |     entityCount = 0;
      | end
      | 
      | % Read the current entity's final time and calculate throughput time
      | entity.EndTime = ReadTime();
      | entity.TTPpackaging = abs(entity.EndTime - entity.EndTimePainting);
      | 
      | % Update the total throughput time and entity count
      | TTPtotal = TTPtotal + entity.TTPpackaging;
      | entityCount = entityCount + 1;
      | 
      | % Calculate the average throughput time
      | avgTTPpackaging = TTPtotal / entityCount;
      | 
      | % Send the average throughput time to the workspace
      | ToWorkspace_Packaging(avgTTPpackaging);
      settings: OutputPortMap=o5,o9
  Packaging with upgrade Upgrade = automated packaging system with vision check DOUBLE UPGRADE extra capacity Process 16 Capacity = 2 : EntityServer  InputPortMessageModes=m  OutputPortMessageModes=n,m  Capacity=1  ServiceTimeSource=MATLAB action  ServiceTimeValue=32  ServiceTimeAction=|  ServiceCompleteAction=|  Utilization=on
      | generateTime = @(mu, cv) lognrnd(log(mu) - 0.5*log(1+cv^2), sqrt(log(1+cv^2)));
      | 
      | dt = generateTime (18.2, 0.65);
      | dt = dt * 0.75;
      | if dt <= 0
      |     dt = 0;
      | end
      | 
      | % Setup times
      | persistent last_product;
      | 
      | if isempty(last_product)
      |     last_product = 0;
      | end
      | 
      | setuptime = 0;
      | 
      | if last_product == 0
      |     % First entity - no setup time needed
      |     setuptime = 0;
      | elseif last_product ~= entity.Product
      |     % Product change detected - apply setup time based on previous product
      |     setuptime = 1;
      | end
      | 
      | dt = dt + setuptime;
      | last_product = entity.Product;
      | % Define persistent variables to track the total throughput time and entity count
      | persistent TTPtotal entityCount;
      | 
      | % Initialize the persistent variables if they are empty
      | if isempty(TTPtotal)
      |     TTPtotal = 0;
      | end
      | if isempty(entityCount)
      |     entityCount = 0;
      | end
      | 
      | % Read the current entity's final time and calculate throughput time
      | entity.EndTime = ReadTime();
      | entity.TTPpackaging = abs(entity.EndTime - entity.EndTimePainting);
      | 
      | % Update the total throughput time and entity count
      | TTPtotal = TTPtotal + entity.TTPpackaging;
      | entityCount = entityCount + 1;
      | 
      | % Calculate the average throughput time
      | avgTTPpackaging = TTPtotal / entityCount;
      | 
      | % Send the average throughput time to the workspace
      | ToWorkspace_Packaging(avgTTPpackaging);
      settings: OutputPortMap=o5,o9
  Painting and Bodywork Process 15 Capacity = 2 : EntityServer  Commented=on  InputPortMessageModes=m  OutputPortMessageModes=n,m  Capacity=2  ServiceTimeSource=MATLAB action  ServiceTimeValue=32  ServiceTimeAction=|  ServiceCompleteAction=|  Utilization=on
      ServiceTimeAction=|
      | if entity.Product == 1 | entity.Product == 2
      |     dt = 30.2;
      | elseif entity.Product == 3 | entity.Product == 4 | entity.Product == 5
      |     dt = 35.4;
      | else
      |     dt = 0;
      | end
      | 
      | % Setup times
      | persistent last_product;
      | 
      | if isempty(last_product)
      |     last_product = 0;
      | end
      | 
      | setuptime = 0;
      | 
      | if last_product == 0
      |     % First entity - no setup time needed
      |     setuptime = 0;
      | elseif last_product ~= entity.Product
      |     % Product change detected - apply setup time based on previous product
      |     setuptime = 2;
      | end
      | 
      | dt = dt + setuptime;
      | last_product = entity.Product;
      ServiceCompleteAction=|
      | % Define persistent variables to track the total throughput time and entity count
      | persistent TTPtotal entityCount;
      | 
      | % Initialize the persistent variables if they are empty
      | if isempty(TTPtotal)
      |     TTPtotal = 0;
      | end
      | if isempty(entityCount)
      |     entityCount = 0;
      | end
      | 
      | % Read the current entity's final time and calculate throughput time
      | entity.EndTimePainting = ReadTime();
      | entity.TTPpainting = abs(entity.EndTimePainting - entity.EndTimeFinalTest);
      | 
      | % Update the total throughput time and entity count
      | TTPtotal = TTPtotal + entity.TTPpainting;
      | entityCount = entityCount + 1;
      | 
      | % Calculate the average throughput time
      | avgTTPpainting = TTPtotal / entityCount;
      | 
      | % Send the average throughput time to the workspace
      | ToWorkspace_Painting(avgTTPpainting);
      settings: OutputPortMap=o5,o9
  Painting and Bodywork with proposed upgrade Upgrade = Integrated 3D scanner Upgrade another traditional painting machine (dt -45%) Process 15 Capacity = 2 : EntityServer  InputPortMessageModes=m  OutputPortMessageModes=n,m  Capacity=2  ServiceTimeSource=MATLAB action  ServiceTimeValue=32  ServiceTimeAction=|  ServiceCompleteAction=|  Utilization=on
      ServiceTimeAction=|
      | if entity.Product == 1 | entity.Product == 3
      |     dt = 30.2 * 0.7 ;
      | elseif entity.Product == 2 | entity.Product == 4 | entity.Product == 5
      |     dt = 35.4 * 0.7 ;
      | else
      |     dt = 0;
      | end
      | 
      | 
      | % Setup times
      | persistent last_product;
      | 
      | if isempty(last_product)
      |     last_product = 0;
      | end
      | 
      | setuptime = 0;
      | 
      | if last_product == 0
      |     % First entity - no setup time needed
      |     setuptime = 0;
      | elseif last_product ~= entity.Product
      |     % Product change detected - apply setup time based on previous product
      |     setuptime = 2;
      | end
      | 
      | dt = dt + setuptime;
      | last_product = entity.Product;
      ServiceCompleteAction=|
      | % Define persistent variables to track the total throughput time and entity count
      | persistent TTPtotal entityCount;
      | 
      | % Initialize the persistent variables if they are empty
      | if isempty(TTPtotal)
      |     TTPtotal = 0;
      | end
      | if isempty(entityCount)
      |     entityCount = 0;
      | end
      | 
      | % Read the current entity's final time and calculate throughput time
      | entity.EndTimePainting = ReadTime();
      | entity.TTPpainting = abs(entity.EndTimePainting - entity.EndTimeFinalTest);
      | 
      | % Update the total throughput time and entity count
      | TTPtotal = TTPtotal + entity.TTPpainting;
      | entityCount = entityCount + 1;
      | 
      | % Calculate the average throughput time
      | avgTTPpainting = TTPtotal / entityCount;
      | 
      | % Send the average throughput time to the workspace
      | ToWorkspace_Painting(avgTTPpainting);
      settings: OutputPortMap=o5,o9
  Painting and Bodywork with proposed upgrade Upgrade = Traditional painting machinie Process 15 Capacity = 2 : EntityServer  Commented=on  InputPortMessageModes=m  OutputPortMessageModes=n,m  Capacity=2  ServiceTimeSource=MATLAB action  ServiceTimeValue=32  ServiceTimeAction=|  ServiceCompleteAction=|  Utilization=on
      ServiceTimeAction=|
      | if entity.Product == 10 | entity.Product == 20
      |     dt = 30.2;
      |     dt = dt * 0.55;
      | elseif entity.Product == 11 | entity.Product == 21 | entity.Product == 35
      |     dt = 35.4;
      |     dt = dt * 0.55;
      | else
      |     dt = 0;
      | end
      ServiceCompleteAction=|
      | % Define persistent variables to track the total throughput time and entity count
      | persistent TTPtotal entityCount;
      | 
      | % Initialize the persistent variables if they are empty
      | if isempty(TTPtotal)
      |     TTPtotal = 0;
      | end
      | if isempty(entityCount)
      |     entityCount = 0;
      | end
      | 
      | % Read the current entity's final time and calculate throughput time
      | entity.EndTimePainting = ReadTime();
      | entity.TTPpainting = abs(entity.EndTimePainting - entity.EndTimeFinalTest);
      | 
      | % Update the total throughput time and entity count
      | TTPtotal = TTPtotal + entity.TTPpainting;
      | entityCount = entityCount + 1;
      | 
      | % Calculate the average throughput time
      | avgTTPpainting = TTPtotal / entityCount;
      | 
      | % Send the average throughput time to the workspace
      | ToWorkspace_Painting(avgTTPpainting);
      settings: OutputPortMap=o5,o9
  Scope{,1..35,42..44,50..51} (41 alike) : Scope
      Scope settings: ActiveDisplayYMinimum=-1494.8749999999998  ActiveDisplayYMaximum=13463.875
      Scope1 settings: ActiveDisplayYMinimum=-3.8745652427469324  ActiveDisplayYMaximum=34.8710871847224
      Scope10 settings: DataLoggingVariableName=ScopeData10
      Scope11 settings: DataLoggingVariableName=ScopeData11
      Scope12 settings: DataLoggingVariableName=ScopeData12
      Scope13 settings: DataLoggingVariableName=ScopeData13
      Scope14 settings: ActiveDisplayYMinimum=-53.85833845332008  ActiveDisplayYMaximum=80.62252617361662  DataLoggingVariableName=ScopeData14
      Scope15 settings: DataLoggingVariableName=ScopeData15
      Scope16 settings: DataLoggingVariableName=ScopeData16
      Scope17 settings: DataLoggingVariableName=ScopeData17
      Scope18 settings: DataLoggingVariableName=ScopeData18
      Scope19 settings: DataLoggingVariableName=ScopeData19
      Scope2 settings: ActiveDisplayYMinimum=-0.12499999999999997  ActiveDisplayYMaximum=1.125  DataLoggingVariableName=ScopeData2
      Scope20 settings: DataLoggingVariableName=ScopeData20
      Scope21 settings: DataLoggingVariableName=ScopeData21
      Scope22 settings: DataLoggingVariableName=ScopeData22
      Scope23 settings: DataLoggingVariableName=ScopeData23
      Scope24 settings: DataLoggingVariableName=ScopeData24
      Scope25 settings: DataLoggingVariableName=ScopeData25  DataLoggingSaveFormat=Array
      Scope26 settings: DataLoggingVariableName=ScopeData26
      Scope27 settings: DataLoggingVariableName=ScopeData27
      Scope28 settings: DataLoggingVariableName=ScopeData28
      Scope29 settings: DataLoggingVariableName=ScopeData29
      Scope3 settings: ActiveDisplayYMinimum=-10.256761124439361  ActiveDisplayYMaximum=27.288569985308015  DataLoggingVariableName=ScopeData3
      Scope30 settings: DataLoggingVariableName=ScopeData30
      Scope31 settings: DataLoggingVariableName=ScopeData31
      Scope32 settings: DataLoggingVariableName=ScopeData32
      Scope33 settings: DataLoggingVariableName=ScopeData33
      Scope34 settings: DataLoggingVariableName=ScopeData34
      Scope35 settings: ActiveDisplayYMinimum=-1  ActiveDisplayYMaximum=1  DataLoggingVariableName=ScopeData35
      Scope4 settings: DataLoggingVariableName=ScopeData4
      Scope42 settings: ActiveDisplayYMinimum=-1  ActiveDisplayYMaximum=1  DataLoggingVariableName=ScopeData42
      Scope43 settings: DataLoggingVariableName=ScopeData43
      Scope44 settings: ActiveDisplayYMinimum=-1  ActiveDisplayYMaximum=1  DataLoggingVariableName=ScopeData44
      Scope5 settings: DataLoggingVariableName=ScopeData5
      Scope50 settings: DataLoggingVariableName=ScopeData50
      Scope51 settings: DataLoggingVariableName=ScopeData51
      Scope6 settings: DataLoggingVariableName=ScopeData6
      Scope7 settings: DataLoggingVariableName=ScopeData7
      Scope8 settings: DataLoggingVariableName=ScopeData8
      Scope9 settings: DataLoggingVariableName=ScopeData9
  Send : Send  OutputPortMessageModes=m
  Send1 : Send  OutputPortMessageModes=m
  Simulink Function : Subsystem  TreatAsAtomicUnit=on
  Simulink Function1 : Subsystem  TreatAsAtomicUnit=on
  Simulink Function10 : Subsystem  TreatAsAtomicUnit=on
  Simulink Function11 : Subsystem  TreatAsAtomicUnit=on
  Simulink Function12 : Subsystem  TreatAsAtomicUnit=on
  Simulink Function2 : Subsystem  TreatAsAtomicUnit=on
  Simulink Function3 : Subsystem  TreatAsAtomicUnit=on
  Simulink Function4 : Subsystem  TreatAsAtomicUnit=on
  Simulink Function5 : Subsystem  TreatAsAtomicUnit=on
  Simulink Function6 : Subsystem  TreatAsAtomicUnit=on
  Simulink Function7 : Subsystem  TreatAsAtomicUnit=on
  Simulink Function8 : Subsystem  TreatAsAtomicUnit=on
  Simulink Function9 : Subsystem  TreatAsAtomicUnit=on
  UtilBoiler : Scope
      settings: ActiveDisplayYMinimum=-1  ActiveDisplayYMaximum=1  DataLoggingVariableName=util_BoilerDept
  UtilChassis : Scope
      settings: ActiveDisplayYMinimum=-1  ActiveDisplayYMaximum=1  DataLoggingVariableName=util_ChassisDept
  UtilComponents : Scope
      settings: ActiveDisplayYMinimum=-1  ActiveDisplayYMaximum=1  DataLoggingVariableName=util_ComponentsDept
  UtilEbox : Scope
      settings: ActiveDisplayYMinimum=-0.18333391237657581  ActiveDisplayYMaximum=1.0081020677583785  DataLoggingVariableName=util_EboxDept
  UtilElec : Scope
      settings: ActiveDisplayYMinimum=-1  ActiveDisplayYMaximum=1  DataLoggingVariableName=util_ElectronicsDept
  UtilElecTest : Scope
      settings: ActiveDisplayYMinimum=-1  ActiveDisplayYMaximum=1  DataLoggingVariableName=util_ElectronicsTest
  UtilFinalTest : Scope
      settings: ActiveDisplayYMinimum=-1  ActiveDisplayYMaximum=1  DataLoggingVariableName=util_FinalTesting
  UtilHydTest : Scope
      settings: ActiveDisplayYMinimum=-1  ActiveDisplayYMaximum=1  DataLoggingVariableName=util_HydraulicsTest
  UtilPackaging : Scope
      settings: ActiveDisplayYMinimum=-1  ActiveDisplayYMaximum=1  DataLoggingVariableName=util_PackagingDept
  UtilPaintingBodywork : Scope
      settings: ActiveDisplayYMinimum=-1  ActiveDisplayYMaximum=1  DataLoggingVariableName=util_PaintBodyDept
  UtilValves : Scope
      settings: ActiveDisplayYMinimum=-1  ActiveDisplayYMaximum=1  DataLoggingVariableName=util_ValvesDept
  Valves Assembly Process 6 and 7 Capacity = 3 : EntityServer  Commented=on  InputPortMessageModes=m  OutputPortMessageModes=n,m  Capacity=3  ServiceTimeSource=MATLAB action  ServiceTimeValue=32  ServiceTimeAction=|  ServiceCompleteAction=|  SortingAttributeName=HydReworked  Utilization=on
      | generateTime = @(mu, cv) lognrnd(log(mu) - 0.5*log(1+cv^2), sqrt(log(1+cv^2)));
      | 
      | if entity.HydReworked == 1
      |     dt = 1;
      | else
      |     if entity.Product == 1
      |     dt = generateTime(40.3, 0.75);
      |     elseif entity.Product == 2
      |     dt = generateTime(41.6, 0.75);
      |     elseif entity.Product == 3
      |     dt = generateTime(39, 0.75) + generateTime(27.3, 0.75);
      |     elseif entity.Product == 4
      |     dt = generateTime(44.2, 0.75) + generateTime(27.3, 0.75);
      |     elseif entity.Product == 5
      |     dt = generateTime(52, 0.75);
      |     else
      |     dt = 0;
      |     end
      | end
      | 
      | % Setup times
      | persistent last_product;
      | 
      | if isempty(last_product)
      |     last_product = 0;
      | end
      | 
      | setuptime = 0;
      | 
      | if last_product == 0
      |     % First entity - no setup time needed
      |     setuptime = 0;
      | elseif last_product ~= entity.Product
      |     % Product change detected - apply setup time based on previous product
      |     if last_product == 1
      |         setuptime = 4;
      |     elseif last_product == 2
      |         setuptime = 4;
      |     elseif last_product == 3
      |         setuptime = 6;
      |     elseif last_product == 4
      |         setuptime = 7;
      |     else
      |         setuptime = 6;
      |     end
      | end
      | 
      | dt = dt + setuptime;
      | last_product = entity.Product;
      | % Define persistent variables to track the total throughput time and entity count
      | persistent TTPtotal entityCount;
      | % TTPtotal = tracks the total TTP of the system. In which, when every new station is visited, the time is added
      | % entityCount =
      | 
      | % Initialize the persistent variables if they are empty
      | if isempty(TTPtotal)
      |     TTPtotal = 0;
      | end
      | if isempty(entityCount)
      |     entityCount = 0;
      | end
      | 
      | % Read the current entity's final time
      | entity.EndTimeValves = ReadTime();
      | 
      | % Calculate the TTP for the chassis department for the specific entity
      | % INCLUDES wait time
      | entity.TTPvalves = abs(entity.EndTimeValves - entity.EndTimeBoiler);
      | 
      | % Update the total throughput time and entity count
      | % This is done AFTER the process, 
      |     % to mark that the entity has gone through the chassis department 
      |         % (thus TTPchassis being added)
      |             % and add that the entity, for each entity after being processed
      |             
      | TTPtotal = TTPtotal + entity.TTPvalves;
      | entityCount = entityCount + 1;
      | 
      | % Calculate the average throughput time for the chassis department
      | avgTTPvalves = TTPtotal / entityCount;
      | 
      | % Send the average throughput time to the workspace
      | ToWorkspace_Valves(avgTTPvalves);
      settings: OutputPortMap=o5,o9
  Valves Assembly Process 6 and 7 Capacity = 4 : EntityServer  InputPortMessageModes=m  OutputPortMessageModes=n,m  Capacity=4  ServiceTimeSource=MATLAB action  ServiceTimeValue=32  ServiceTimeAction=|  ServiceCompleteAction=|  SortingAttributeName=HydReworked  Utilization=on
      | generateTime = @(mu, cv) lognrnd(log(mu) - 0.5*log(1+cv^2), sqrt(log(1+cv^2)));
      | 
      | if entity.HydReworked == 1
      |     dt = 1;
      | else
      |     if entity.Product == 1
      |     dt = generateTime(40.3, 0.75);
      |     elseif entity.Product == 3
      |     dt = generateTime(41.6, 0.75);
      |     elseif entity.Product == 2
      |     dt = generateTime(39, 0.75) + generateTime(27.3, 0.75);
      |     elseif entity.Product == 4
      |     dt = generateTime(44.2, 0.75) + generateTime(27.3, 0.75);
      |     elseif entity.Product == 5
      |     dt = generateTime(52, 0.75);
      |     else
      |     dt = 0;
      |     end
      | end
      | 
      | % Setup times
      | persistent last_product;
      | 
      | if isempty(last_product)
      |     last_product = 0;
      | end
      | 
      | setuptime = 0;
      | 
      | if last_product == 0
      |     % First entity - no setup time needed
      |     setuptime = 0;
      | elseif last_product ~= entity.Product
      |     % Product change detected - apply setup time based on previous product
      |     if last_product == 1
      |         setuptime = 4;
      |     elseif last_product == 2
      |         setuptime = 4;
      |     elseif last_product == 3
      |         setuptime = 6;
      |     elseif last_product == 4
      |         setuptime = 7;
      |     else
      |         setuptime = 6;
      |     end
      | end
      | 
      | dt = dt + setuptime;
      | last_product = entity.Product;
      | % Define persistent variables to track the total throughput time and entity count
      | persistent TTPtotal entityCount;
      | % TTPtotal = tracks the total TTP of the system. In which, when every new station is visited, the time is added
      | % entityCount =
      | 
      | % Initialize the persistent variables if they are empty
      | if isempty(TTPtotal)
      |     TTPtotal = 0;
      | end
      | if isempty(entityCount)
      |     entityCount = 0;
      | end
      | 
      | % Read the current entity's final time
      | entity.EndTimeValves = ReadTime();
      | 
      | % Calculate the TTP for the chassis department for the specific entity
      | % INCLUDES wait time
      | entity.TTPvalves = abs(entity.EndTimeValves - entity.EndTimeBoiler);
      | 
      | % Update the total throughput time and entity count
      | % This is done AFTER the process, 
      |     % to mark that the entity has gone through the chassis department 
      |         % (thus TTPchassis being added)
      |             % and add that the entity, for each entity after being processed
      |             
      | TTPtotal = TTPtotal + entity.TTPvalves;
      | entityCount = entityCount + 1;
      | 
      | % Calculate the average throughput time for the chassis department
      | avgTTPvalves = TTPtotal / entityCount;
      | 
      | % Send the average throughput time to the workspace
      | ToWorkspace_Valves(avgTTPvalves);
      settings: OutputPortMap=o5,o9
  wires:
  Entity Generator Proposed Solution on Boiler Assembly Reduces defects (rework and scrap) by 20% HAS TO BE PAIRED WITH ENTITY SERVER/1 -> Gain/1, Scope/1
  Entity Queue/3 -> Scope1/1
  Entity Queue/2 -> Scope2/1
  Entity Queue/1 -> Scope3/1
  Entity Queue10/4 -> Entity Gate1/2
  Entity Queue6/4 -> Entity Input Switch/2
  Entity Queue6/1 -> Scope12/1
  Entity Queue6/3 -> Scope11/1
  Entity Queue6/2 -> Scope10/1
  Send/1 -> Entity Gate1/1
  From Workspace/1 -> Send/1
  Entity Queue10/3 -> Scope13/1
  Entity Queue10/2 -> Scope14/1
  Entity Queue10/1 -> Scope15/1
  Entity Queue1/3 -> Scope16/1
  Entity Queue1/2 -> Scope17/1
  Entity Queue1/1 -> Scope18/1
  Entity Output Switch/3 -> Entity Terminator/1
  Entity Output Switch/1 -> Entity Queue3/1
  Entity Output Switch/2 -> Entity Server/1
  Entity Queue3/3 -> Scope6/1
  Entity Queue3/2 -> Scope4/1
  Entity Queue3/1 -> Scope5/1
  Entity Server/1 -> Scope7/1
  Entity Queue2/3 -> Scope8/1
  Entity Queue2/2 -> Scope9/1
  Entity Queue2/1 -> Scope19/1
  Entity Queue3/4 -> Entity Input Switch1/2
  Entity Output Switch1/2 -> Entity Server1/1
  Entity Queue4/3 -> Scope20/1
  Entity Queue4/2 -> Scope21/1
  Entity Queue4/1 -> Scope22/1
  Entity Output Switch1/1 -> Entity Queue5/1
  Entity Output Switch1/3 -> Entity Terminator1/1
  Entity Queue5/4 -> Entity Input Switch2/2
  Entity Output Switch2/2 -> Entity Server2/1
  Entity Output Switch2/3 -> Entity Terminator2/1
  Entity Output Switch2/1 -> Entity Queue8/1
  Entity Queue5/3 -> Scope23/1
  Entity Queue5/2 -> Scope24/1
  Entity Queue5/1 -> Scope25/1
  Entity Queue7/3 -> Scope26/1
  Entity Queue7/2 -> Scope27/1
  Entity Queue7/1 -> Scope28/1
  Entity Queue8/3 -> Scope29/1
  Entity Queue8/1 -> Scope30/1
  Entity Queue8/2 -> Scope31/1
  Entity Queue8/4 -> Entity Gate/2
  Send1/1 -> Entity Gate/1
  From Workspace1/1 -> Send1/1
  Entity Queue9/3 -> Scope32/1
  Entity Queue9/2 -> Scope33/1
  Entity Queue9/1 -> Scope34/1
  Entity Server/2 -> Entity Queue11/1
  Entity Queue11/1 -> Entity Input Switch/1
  Entity Server1/2 -> Entity Queue12/1
  Entity Queue12/1 -> Entity Input Switch1/1
  Entity Server2/2 -> Entity Queue13/1
  Entity Queue13/1 -> Entity Input Switch2/1
  Entity Terminator/1 -> Gain1/1, Scope42/1
  Entity Terminator1/1 -> Gain2/1, Scope43/1
  Entity Terminator2/1 -> Gain3/1, Scope44/1
  Entity Server1/1 -> Scope50/1
  Entity Server2/1 -> Scope51/1
  Entity Output Switch3/1 -> Entity Terminator3/1
  Entity Output Switch3/2 -> Entity Terminator4/1
  Entity Output Switch3/3 -> Entity Terminator5/1
  Entity Output Switch3/4 -> Entity Terminator6/1
  Entity Output Switch3/5 -> Entity Terminator7/1
  Entity Terminator3/1 -> Display/1, Gain4/1
  Entity Terminator4/1 -> Gain8/1, Display1/1
  Entity Terminator5/1 -> Gain7/1, Display2/1
  Entity Terminator6/1 -> Gain6/1, Display3/1
  Entity Terminator7/1 -> Gain5/1, Display4/1
  Gain/1 -> Add/1
  Gain1/1 -> Add/2
  Gain2/1 -> Add/3
  Gain3/1 -> Add/4
  Gain4/1 -> Add/5
  Add/1 -> Display5/1
  Gain8/1 -> Add/6
  Gain7/1 -> Add/7
  Gain6/1 -> Add/8
  Gain5/1 -> Add/9
  Entity Generator Proposed Solution on Boiler Assembly Reduces defects (rework and scrap) by 20% HAS TO BE PAIRED WITH ENTITY SERVER/2 -> Entity Replicator/1
  Additional Time Based on the last entity type Models the setup time after batches/2 -> Entity Queue/1
  Additional Time Based on the last entity type Models the setup time after batches/1 -> Scope35/1
  Entity Replicator/1 -> Additional Time Based on the last entity type Models the setup time after batches/1
  Entity Replicator/2 -> Entity Terminator8/1
  Hydraulics Testing with proposed upgrade Upgrade = Automated parallel multimachine hyd testing cell DOUBLE upgrade AI optimized testing routines Process 8 Capacity = 2/2 -> Entity Output Switch/1
  Entity Queue2/4 -> Hydraulics Testing with proposed upgrade Upgrade = Automated parallel multimachine hyd testing cell DOUBLE upgrade AI optimized testing routines Process 8 Capacity = 2/1
  Hydraulics Testing with proposed upgrade Upgrade = Automated parallel multimachine hyd testing cell DOUBLE upgrade AI optimized testing routines Process 8 Capacity = 2/1 -> UtilHydTest/1
  Entity Queue/4 -> Chassis Assembly with proposed upgrade Upgrade = collaborative robot with force feedback for main chassis ADDITIONAL WORKBENCH ADDED Process 1 and 2 Capacity = 3 machines1/1
  Chassis Assembly with proposed upgrade Upgrade = collaborative robot with force feedback for main chassis ADDITIONAL WORKBENCH ADDED Process 1 and 2 Capacity = 3 machines1/2 -> Entity Queue10/1
  Chassis Assembly with proposed upgrade Upgrade = collaborative robot with force feedback for main chassis ADDITIONAL WORKBENCH ADDED Process 1 and 2 Capacity = 3 machines1/1 -> UtilChassis/1
  Entity Gate1/1 -> Electrical Box Assembly with proposed upgrade Upgrade = Additional assembly station Process 3 Capacity = 2 machine1/1
  Electrical Box Assembly with proposed upgrade Upgrade = Additional assembly station Process 3 Capacity = 2 machine1/2 -> Entity Queue6/1
  Electrical Box Assembly with proposed upgrade Upgrade = Additional assembly station Process 3 Capacity = 2 machine1/1 -> UtilEbox/1
  Entity Queue1/4 -> Valves Assembly Process 6 and 7 Capacity = 4/1
  Valves Assembly Process 6 and 7 Capacity = 4/2 -> Entity Queue2/1
  Valves Assembly Process 6 and 7 Capacity = 4/1 -> UtilValves/1
  Boiler Assembly with proposed upgrade Upgrade = Vision-guided robot for main boiler insertion DOUBLE UPGRADE with AR based assembly TRIPLE upgrade insertion robot Process 4 and 5/1 -> UtilBoiler/1
  Entity Input Switch/1 -> Boiler Assembly with proposed upgrade Upgrade = Vision-guided robot for main boiler insertion DOUBLE UPGRADE with AR based assembly TRIPLE upgrade insertion robot Process 4 and 5/1
  Boiler Assembly with proposed upgrade Upgrade = Vision-guided robot for main boiler insertion DOUBLE UPGRADE with AR based assembly TRIPLE upgrade insertion robot Process 4 and 5/2 -> Entity Queue1/1
  Components Assembly with proposed upgrade Upgrade = collaborative robot Process 12 and 13 Capacity = 1/2 -> Entity Queue7/1
  Entity Input Switch2/1 -> Components Assembly with proposed upgrade Upgrade = collaborative robot Process 12 and 13 Capacity = 1/1
  Components Assembly with proposed upgrade Upgrade = collaborative robot Process 12 and 13 Capacity = 1/1 -> UtilComponents/1
  Entity Queue9/4 -> Packaging with upgrade Upgrade = automated packaging system with vision check DOUBLE UPGRADE extra capacity Process 16 Capacity = 2/1
  Packaging with upgrade Upgrade = automated packaging system with vision check DOUBLE UPGRADE extra capacity Process 16 Capacity = 2/2 -> Entity Output Switch3/1
  Packaging with upgrade Upgrade = automated packaging system with vision check DOUBLE UPGRADE extra capacity Process 16 Capacity = 2/1 -> UtilPackaging/1
  Entity Gate/1 -> Painting and Bodywork with proposed upgrade Upgrade = Integrated 3D scanner Upgrade another traditional painting machine (dt -45%) Process 15 Capacity = 2/1
  Painting and Bodywork with proposed upgrade Upgrade = Integrated 3D scanner Upgrade another traditional painting machine (dt -45%) Process 15 Capacity = 2/2 -> Entity Queue9/1
  Painting and Bodywork with proposed upgrade Upgrade = Integrated 3D scanner Upgrade another traditional painting machine (dt -45%) Process 15 Capacity = 2/1 -> UtilPaintingBodywork/1
  Electronics Assembly with proposed upgrade Upgrade = Display mounting assist system DOUBLE UPGRADE extra capacity Process 9 and 10/2 -> Entity Queue4/1
  Entity Input Switch1/1 -> Electronics Assembly with proposed upgrade Upgrade = Display mounting assist system DOUBLE UPGRADE extra capacity Process 9 and 10/1
  Electronics Assembly with proposed upgrade Upgrade = Display mounting assist system DOUBLE UPGRADE extra capacity Process 9 and 10/1 -> UtilElec/1
  Entity Queue4/4 -> Electronics Testing with proposed upgrade Upgrade = Automated CPU burn-in testing Impact = Test time -20% Process 11 Capacity = 1/1
  Electronics Testing with proposed upgrade Upgrade = Automated CPU burn-in testing Impact = Test time -20% Process 11 Capacity = 1/2 -> Entity Output Switch1/1
  Electronics Testing with proposed upgrade Upgrade = Automated CPU burn-in testing Impact = Test time -20% Process 11 Capacity = 1/1 -> UtilElecTest/1
  Final testing with proposed upgrade Upgrade = AI optimized testing routines DOUBLE UPGRADE enhanced station Process 14 Capacity = 2/1 -> UtilFinalTest/1
  Entity Queue7/4 -> Final testing with proposed upgrade Upgrade = AI optimized testing routines DOUBLE UPGRADE enhanced station Process 14 Capacity = 2/1
  Final testing with proposed upgrade Upgrade = AI optimized testing routines DOUBLE UPGRADE enhanced station Process 14 Capacity = 2/2 -> Entity Output Switch2/1
  Final Testing Process 14 Capacity = 1/2 -> Packaging Process 16 Capacity = Upgraded/1
